simulink model "model"  (R2014a)
(part 4 of 5)

  Ajka___Sümeg_CN_190281225_120000_CN_209328058_120000/RConn2 -- T_209328058__Zalaegerszeg_alállomás/LConn2 -- _CN_312831631_120000_CN_209328058_120000/LConn2
  Ajka___Sümeg_CN_190281225_120000_CN_209328058_120000/RConn3 -- T_209328058__Zalaegerszeg_alállomás/LConn3 -- _CN_312831631_120000_CN_209328058_120000/LConn3 -- bus22/LConn1
  Ajka___Sümeg_CN_190281225_120000_CN_243983151_120000/RConn1 -- T_243983151_120000;11000_Keszthely_alállomás/LConn1 -- Söjtör___Keszthely_CN_243983151_120000_CN_203404634_120000/LConn1 -- Söjtör___Keszthely_CN_243983151_120000_CN_243816689_120000/LConn1 -- Keszthely___Marcali_CN_243983151_120000_CN_311788820_120000/LConn1 -- _CN_243983151_120000_CN_65034002_120000/RConn1 -- _CN_243983151_120000_CN_234435878_120000/LConn1 -- _CN_243983151_120000_CN_170160989_120000/LConn1 -- Keszthely–Hévíz_CN_96705565_120000_CN_243983151_120000/LConn1
  Ajka___Sümeg_CN_190281225_120000_CN_243983151_120000/RConn2 -- T_243983151_120000;11000_Keszthely_alállomás/LConn2 -- Söjtör___Keszthely_CN_243983151_120000_CN_203404634_120000/LConn2 -- Söjtör___Keszthely_CN_243983151_120000_CN_243816689_120000/LConn2 -- Keszthely___Marcali_CN_243983151_120000_CN_311788820_120000/LConn2 -- _CN_243983151_120000_CN_65034002_120000/RConn2 -- _CN_243983151_120000_CN_234435878_120000/LConn2 -- _CN_243983151_120000_CN_170160989_120000/LConn2 -- Keszthely–Hévíz_CN_96705565_120000_CN_243983151_120000/LConn2
  Ajka___Sümeg_CN_190281225_120000_CN_243983151_120000/RConn3 -- T_243983151_120000;11000_Keszthely_alállomás/LConn3 -- Söjtör___Keszthely_CN_243983151_120000_CN_203404634_120000/LConn3 -- Söjtör___Keszthely_CN_243983151_120000_CN_243816689_120000/LConn3 -- bus23/LConn1 -- Keszthely___Marcali_CN_243983151_120000_CN_311788820_120000/LConn3 -- _CN_243983151_120000_CN_65034002_120000/RConn3 -- _CN_243983151_120000_CN_234435878_120000/LConn3 -- _CN_243983151_120000_CN_170160989_120000/LConn3 -- Keszthely–Hévíz_CN_96705565_120000_CN_243983151_120000/LConn3
  T_167473416__/LConn1 -- Ajka___Sümeg_CN_190281225_120000_CN_167473416_120000/RConn1
  T_167473416__/LConn2 -- Ajka___Sümeg_CN_190281225_120000_CN_167473416_120000/RConn2
  Ajka___Sümeg_CN_190281225_120000_CN_167473416_120000/RConn3 -- T_167473416__/LConn3 -- bus24/LConn1
  Ajka___Sümeg_CN_190281225_120000_CN_320532045_120000/RConn1 -- T_320532045__Ajka/LConn1 -- Ajka–Litér_CN_320532045_120000_CN_65034002_120000/RConn1 -- Ikervár___Celldömölk;_Szombathely–Ajka_CN_180089895_120000_CN_320532045_120000/LConn1 -- Pápa–Ajka_CN_320532045_120000_CN_313625037_120000/LConn1
  Ajka___Sümeg_CN_190281225_120000_CN_320532045_120000/RConn2 -- T_320532045__Ajka/LConn2 -- Ajka–Litér_CN_320532045_120000_CN_65034002_120000/RConn2 -- Ikervár___Celldömölk;_Szombathely–Ajka_CN_180089895_120000_CN_320532045_120000/LConn2 -- Pápa–Ajka_CN_320532045_120000_CN_313625037_120000/LConn2
  Ajka___Sümeg_CN_190281225_120000_CN_320532045_120000/RConn3 -- T_320532045__Ajka/LConn3 -- Ajka–Litér_CN_320532045_120000_CN_65034002_120000/RConn3 -- bus25/LConn1 -- Ikervár___Celldömölk;_Szombathely–Ajka_CN_180089895_120000_CN_320532045_120000/LConn3 -- Pápa–Ajka_CN_320532045_120000_CN_313625037_120000/LConn3
  _CN_299594250_120000_CN_299717539_120000/LConn1 -- T_299594250__/LConn1 -- _CN_299594250_120000_CN_301002581_120000/LConn1 -- _CN_299594250_120000_CN_299717558_120000/LConn1
  _CN_299594250_120000_CN_299717539_120000/LConn2 -- T_299594250__/LConn2 -- _CN_299594250_120000_CN_301002581_120000/LConn2 -- _CN_299594250_120000_CN_299717558_120000/LConn2
  _CN_299594250_120000_CN_299717539_120000/LConn3 -- T_299594250__/LConn3 -- _CN_299594250_120000_CN_301002581_120000/LConn3 -- _CN_299594250_120000_CN_299717558_120000/LConn3 -- bus26/LConn1
  _CN_299594250_120000_CN_299717539_120000/RConn1 -- T_299717539__/LConn1 -- _CN_173757619_120000_CN_299717539_120000/LConn1
  _CN_299594250_120000_CN_299717539_120000/RConn2 -- T_299717539__/LConn2 -- _CN_173757619_120000_CN_299717539_120000/LConn2
  _CN_299594250_120000_CN_299717539_120000/RConn3 -- T_299717539__/LConn3 -- _CN_173757619_120000_CN_299717539_120000/LConn3 -- bus27/LConn1
  _CN_299594250_120000_CN_301002581_120000/RConn1 -- T_301002581__/RConn1 -- _CN_104027708_120000_CN_301002581_120000/LConn1 -- Nagybátony_Mátravidéki_Erőmű_CN_173757619_120000_CN_301002581_120000/LConn1 -- L_301002581/LConn1
  _CN_299594250_120000_CN_301002581_120000/RConn2 -- T_301002581__/RConn2 -- _CN_104027708_120000_CN_301002581_120000/LConn2 -- Nagybátony_Mátravidéki_Erőmű_CN_173757619_120000_CN_301002581_120000/LConn2 -- L_301002581/LConn2
  _CN_299594250_120000_CN_301002581_120000/RConn3 -- T_301002581__/RConn3 -- _CN_104027708_120000_CN_301002581_120000/LConn3 -- Nagybátony_Mátravidéki_Erőmű_CN_173757619_120000_CN_301002581_120000/LConn3 -- L_301002581/LConn3 -- bus28/LConn1
  T_299717558__Rétság_alállomás/LConn1 -- _CN_299594250_120000_CN_299717558_120000/RConn1
  T_299717558__Rétság_alállomás/LConn2 -- _CN_299594250_120000_CN_299717558_120000/RConn2
  _CN_299594250_120000_CN_299717558_120000/RConn3 -- T_299717558__Rétság_alállomás/LConn3 -- bus29/LConn1
  Csurgó–Nagyatád_CN_167798796_120000_CN_31538924_120000/LConn1 -- T_167798796__Nagyatád_alállomás/LConn1 -- Csurgó–Nagyatád_CN_167798796_120000_CN_244495956_120000/LConn1 -- Csurgó–Nagyatád_CN_167798796_120000_CN_203404634_120000/LConn1 -- Csurgó–Nagyatád_CN_167798796_120000_CN_121241890_120000/LConn1
  Csurgó–Nagyatád_CN_167798796_120000_CN_31538924_120000/LConn2 -- T_167798796__Nagyatád_alállomás/LConn2 -- Csurgó–Nagyatád_CN_167798796_120000_CN_244495956_120000/LConn2 -- Csurgó–Nagyatád_CN_167798796_120000_CN_203404634_120000/LConn2 -- Csurgó–Nagyatád_CN_167798796_120000_CN_121241890_120000/LConn2
  Csurgó–Nagyatád_CN_167798796_120000_CN_31538924_120000/LConn3 -- T_167798796__Nagyatád_alállomás/LConn3 -- Csurgó–Nagyatád_CN_167798796_120000_CN_244495956_120000/LConn3 -- Csurgó–Nagyatád_CN_167798796_120000_CN_203404634_120000/LConn3 -- bus30/LConn1 -- Csurgó–Nagyatád_CN_167798796_120000_CN_121241890_120000/LConn3
  Csurgó–Nagyatád_CN_167798796_120000_CN_31538924_120000/RConn1 -- T_31538924__Kaposvár_alállomás/LConn1 -- Pécsi_Hőerőmű–(Bonyhád_–_Szekszárd_–_Paks)_Komló_CN_302192173_120000_CN_31538924_120000/LConn1 -- _CN_311788819_120000_CN_31538924_120000/LConn1 -- Kaposvár–Kaposfüred_CN_315669517_120000_CN_31538924_120000/LConn1 -- Kaposvár_–_Sikonda_CN_235409083_120000_CN_31538924_120000/LConn1 -- Kaposvár–Toponár_CN_31538924_120000_CN_113570302_120000/LConn1
  Csurgó–Nagyatád_CN_167798796_120000_CN_31538924_120000/RConn2 -- T_31538924__Kaposvár_alállomás/LConn2 -- Pécsi_Hőerőmű–(Bonyhád_–_Szekszárd_–_Paks)_Komló_CN_302192173_120000_CN_31538924_120000/LConn2 -- _CN_311788819_120000_CN_31538924_120000/LConn2 -- Kaposvár–Kaposfüred_CN_315669517_120000_CN_31538924_120000/LConn2 -- Kaposvár_–_Sikonda_CN_235409083_120000_CN_31538924_120000/LConn2 -- Kaposvár–Toponár_CN_31538924_120000_CN_113570302_120000/LConn2
  Csurgó–Nagyatád_CN_167798796_120000_CN_31538924_120000/RConn3 -- T_31538924__Kaposvár_alállomás/LConn3 -- Pécsi_Hőerőmű–(Bonyhád_–_Szekszárd_–_Paks)_Komló_CN_302192173_120000_CN_31538924_120000/LConn3 -- _CN_311788819_120000_CN_31538924_120000/LConn3 -- Kaposvár–Kaposfüred_CN_315669517_120000_CN_31538924_120000/LConn3 -- Kaposvár_–_Sikonda_CN_235409083_120000_CN_31538924_120000/LConn3 -- Kaposvár–Toponár_CN_31538924_120000_CN_113570302_120000/LConn3 -- bus31/LConn1
  Csurgó–Nagyatád_CN_167798796_120000_CN_121241890_120000/RConn1 -- T_121241890__Szigetvár_120_kV_alállomás/LConn1 -- Kővágószőlős–Szigetvár_CN_121241890_120000_CN_313889220_120000/LConn1 -- Barcs___Szigetvár_120_Kv_s_távvezeték_CN_121241890_120000_CN_121135019_120000/LConn1
  Csurgó–Nagyatád_CN_167798796_120000_CN_121241890_120000/RConn2 -- T_121241890__Szigetvár_120_kV_alállomás/LConn2 -- Kővágószőlős–Szigetvár_CN_121241890_120000_CN_313889220_120000/LConn2 -- Barcs___Szigetvár_120_Kv_s_távvezeték_CN_121241890_120000_CN_121135019_120000/LConn2
  Csurgó–Nagyatád_CN_167798796_120000_CN_121241890_120000/RConn3 -- T_121241890__Szigetvár_120_kV_alállomás/LConn3 -- Kővágószőlős–Szigetvár_CN_121241890_120000_CN_313889220_120000/LConn3 -- bus32/LConn1 -- Barcs___Szigetvár_120_Kv_s_távvezeték_CN_121241890_120000_CN_121135019_120000/LConn3
  T_244495956__Csurgó_alállomás/LConn1 -- Csurgó–Nagyatád_CN_167798796_120000_CN_244495956_120000/RConn1
  T_244495956__Csurgó_alállomás/LConn2 -- Csurgó–Nagyatád_CN_167798796_120000_CN_244495956_120000/RConn2
  Csurgó–Nagyatád_CN_167798796_120000_CN_244495956_120000/RConn3 -- T_244495956__Csurgó_alállomás/LConn3 -- bus33/LConn1
  Csurgó–Nagyatád_CN_167798796_120000_CN_203404634_120000/RConn1 -- T_203404634_120000;20000;10000_Nagykanizsa_alállomás/LConn1 -- Söjtör___Keszthely_CN_243983151_120000_CN_203404634_120000/RConn1 -- Kanizsavár___Nagykanizsa_CN_203404634_120000_CN_243726196_120000/LConn1
  Csurgó–Nagyatád_CN_167798796_120000_CN_203404634_120000/RConn2 -- T_203404634_120000;20000;10000_Nagykanizsa_alállomás/LConn2 -- Söjtör___Keszthely_CN_243983151_120000_CN_203404634_120000/RConn2 -- Kanizsavár___Nagykanizsa_CN_203404634_120000_CN_243726196_120000/LConn2
  Csurgó–Nagyatád_CN_167798796_120000_CN_203404634_120000/RConn3 -- T_203404634_120000;20000;10000_Nagykanizsa_alállomás/LConn3 -- Söjtör___Keszthely_CN_243983151_120000_CN_203404634_120000/RConn3 -- Kanizsavár___Nagykanizsa_CN_203404634_120000_CN_243726196_120000/LConn3 -- bus34/LConn1
  _CN_254851597_120000_CN_254847446_120000/LConn1 -- T_254851597__Bicske_alállomás/LConn1 -- _CN_254851597_120000_CN_254910050_120000/RConn1
  _CN_254851597_120000_CN_254847446_120000/LConn2 -- T_254851597__Bicske_alállomás/LConn2 -- _CN_254851597_120000_CN_254910050_120000/RConn2
  _CN_254851597_120000_CN_254847446_120000/LConn3 -- T_254851597__Bicske_alállomás/LConn3 -- _CN_254851597_120000_CN_254910050_120000/RConn3 -- bus35/LConn1
  _CN_254851597_120000_CN_254847446_120000/RConn1 -- T_254847446__Bicske_dél_alállomás/RConn1 -- _CN_153098964_120000_CN_254847446_120000/LConn1 -- L_254847446/LConn1
  _CN_254851597_120000_CN_254847446_120000/RConn2 -- T_254847446__Bicske_dél_alállomás/RConn2 -- _CN_153098964_120000_CN_254847446_120000/LConn2 -- L_254847446/LConn2
  _CN_254851597_120000_CN_254847446_120000/RConn3 -- T_254847446__Bicske_dél_alállomás/RConn3 -- _CN_153098964_120000_CN_254847446_120000/LConn3 -- L_254847446/LConn3 -- bus36/LConn1
  T_350686736__Győr_Dunapart_alállomás/LConn1 -- _CN_350686736_120000_CN_350230665_120000/LConn1
  T_350686736__Győr_Dunapart_alállomás/LConn2 -- _CN_350686736_120000_CN_350230665_120000/LConn2
  _CN_350686736_120000_CN_350230665_120000/LConn3 -- T_350686736__Győr_Dunapart_alállomás/LConn3 -- bus37/LConn1
  _CN_350686736_120000_CN_350230665_120000/RConn1 -- T_350230665__Győr_ÉDÁSZ_alállomás/LConn1 -- _CN_124244078_120000_CN_350230665_120000/LConn1 -- _CN_267155016_120000_CN_350230665_120000/LConn1
  _CN_350686736_120000_CN_350230665_120000/RConn2 -- T_350230665__Győr_ÉDÁSZ_alállomás/LConn2 -- _CN_124244078_120000_CN_350230665_120000/LConn2 -- _CN_267155016_120000_CN_350230665_120000/LConn2
  _CN_350686736_120000_CN_350230665_120000/RConn3 -- T_350230665__Győr_ÉDÁSZ_alállomás/LConn3 -- _CN_124244078_120000_CN_350230665_120000/LConn3 -- bus38/LConn1 -- _CN_267155016_120000_CN_350230665_120000/LConn3
  T_288399377__Szeged_Cserepes_sori_alállomás/LConn1 -- _CN_288399377_120000_CN_111678830_120000/LConn1
  T_288399377__Szeged_Cserepes_sori_alállomás/LConn2 -- _CN_288399377_120000_CN_111678830_120000/LConn2
  _CN_288399377_120000_CN_111678830_120000/LConn3 -- T_288399377__Szeged_Cserepes_sori_alállomás/LConn3 -- bus39/LConn1
  _CN_288399377_120000_CN_111678830_120000/RConn1 -- T_111678830__Szeged_alállomás/RConn1 -- Szeged___Sándorfalva_CN_100962927_120000_CN_111678830_120000/LConn1 -- L_111678830/LConn1
  _CN_288399377_120000_CN_111678830_120000/RConn2 -- T_111678830__Szeged_alállomás/RConn2 -- Szeged___Sándorfalva_CN_100962927_120000_CN_111678830_120000/LConn2 -- L_111678830/LConn2
  _CN_288399377_120000_CN_111678830_120000/RConn3 -- T_111678830__Szeged_alállomás/RConn3 -- Szeged___Sándorfalva_CN_100962927_120000_CN_111678830_120000/LConn3 -- L_111678830/LConn3 -- bus40/LConn1
  T_296680978__/LConn1 -- _CN_296680978_120000_CN_119367515_120000/LConn1
  T_296680978__/LConn2 -- _CN_296680978_120000_CN_119367515_120000/LConn2
  _CN_296680978_120000_CN_119367515_120000/LConn3 -- T_296680978__/LConn3 -- bus41/LConn1
  T_119367515__/LConn1 -- _CN_296680978_120000_CN_119367515_120000/RConn1
  T_119367515__/LConn2 -- _CN_296680978_120000_CN_119367515_120000/RConn2
  _CN_296680978_120000_CN_119367515_120000/RConn3 -- T_119367515__/LConn3 -- bus42/LConn1
  T_251991299_220000;120000_Detk_220_120_kV_os_alállomás/LConn1 -- Nagybátony___Detk_CN_251991299_120000_CN_173757619_120000/LConn1
  T_251991299_220000;120000_Detk_220_120_kV_os_alállomás/LConn2 -- Nagybátony___Detk_CN_251991299_120000_CN_173757619_120000/LConn2
  Nagybátony___Detk_CN_251991299_120000_CN_173757619_120000/LConn3 -- T_251991299_220000;120000_Detk_220_120_kV_os_alállomás/LConn3 -- bus43/LConn1
  Nagybátony___Detk_CN_251991299_120000_CN_173757619_120000/RConn1 -- T_173757619__Nagybátony_alállomás/LConn1 -- _CN_173757619_120000_CN_299717539_120000/RConn1 -- Salgótarján_Öntöde_–_Nagybátony_CN_173757619_120000_CN_355349327_120000/LConn1 -- Nagybátony_Mátravidéki_Erőmű_CN_173757619_120000_CN_301002581_120000/RConn1 -- Nagybátony___Borsodnádasd_CN_173757619_120000_CN_302147975_120000/LConn1
  Nagybátony___Detk_CN_251991299_120000_CN_173757619_120000/RConn2 -- T_173757619__Nagybátony_alállomás/LConn2 -- _CN_173757619_120000_CN_299717539_120000/RConn2 -- Salgótarján_Öntöde_–_Nagybátony_CN_173757619_120000_CN_355349327_120000/LConn2 -- Nagybátony_Mátravidéki_Erőmű_CN_173757619_120000_CN_301002581_120000/RConn2 -- Nagybátony___Borsodnádasd_CN_173757619_120000_CN_302147975_120000/LConn2
  Nagybátony___Detk_CN_251991299_120000_CN_173757619_120000/RConn3 -- T_173757619__Nagybátony_alállomás/LConn3 -- _CN_173757619_120000_CN_299717539_120000/RConn3 -- Salgótarján_Öntöde_–_Nagybátony_CN_173757619_120000_CN_355349327_120000/LConn3 -- Nagybátony_Mátravidéki_Erőmű_CN_173757619_120000_CN_301002581_120000/RConn3 -- bus44/LConn1 -- Nagybátony___Borsodnádasd_CN_173757619_120000_CN_302147975_120000/LConn3
  T_299574805__/LConn1 -- _CN_299574805_120000_CN_252028146_120000/LConn1
  T_299574805__/LConn2 -- _CN_299574805_120000_CN_252028146_120000/LConn2
  _CN_299574805_120000_CN_252028146_120000/LConn3 -- T_299574805__/LConn3 -- bus45/LConn1
  _CN_299574805_120000_CN_252028146_120000/RConn1 -- T_252028146_220000;120000;12000_Szolnok_220_120_20_kV_os_Alállomás/RConn4 -- _CN_252028146_120000_CN_289011848_120000/LConn1 -- _CN_252028146_120000_CN_288863210_120000/LConn1 -- L_252028146/LConn1 -- Tiszakécske–Városföld_CN_281553159_120000_CN_252028146_120000/LConn1 -- _CN_321513575_120000_CN_252028146_120000/LConn1 -- Szolnok–Cegléd_CN_223956685_120000_CN_252028146_120000/LConn1
  _CN_299574805_120000_CN_252028146_120000/RConn2 -- T_252028146_220000;120000;12000_Szolnok_220_120_20_kV_os_Alállomás/RConn5 -- _CN_252028146_120000_CN_289011848_120000/LConn2 -- _CN_252028146_120000_CN_288863210_120000/LConn2 -- L_252028146/LConn2 -- Tiszakécske–Városföld_CN_281553159_120000_CN_252028146_120000/LConn2 -- _CN_321513575_120000_CN_252028146_120000/LConn2 -- Szolnok–Cegléd_CN_223956685_120000_CN_252028146_120000/LConn2
  _CN_299574805_120000_CN_252028146_120000/RConn3 -- T_252028146_220000;120000;12000_Szolnok_220_120_20_kV_os_Alállomás/RConn6 -- _CN_252028146_120000_CN_289011848_120000/LConn3 -- _CN_252028146_120000_CN_288863210_120000/LConn3 -- L_252028146/LConn3 -- bus46/LConn1 -- Tiszakécske–Városföld_CN_281553159_120000_CN_252028146_120000/LConn3 -- _CN_321513575_120000_CN_252028146_120000/LConn3 -- Szolnok–Cegléd_CN_223956685_120000_CN_252028146_120000/LConn3
  Keszthely–Hévíz_CN_96705565_120000_CN_243983151_120000/RConn1 -- T_96705565_400000;120000_Hévíz_400_120_kV_alállomás/RConn1 -- L_96705565/LConn1
  Keszthely–Hévíz_CN_96705565_120000_CN_243983151_120000/RConn2 -- T_96705565_400000;120000_Hévíz_400_120_kV_alállomás/RConn2 -- L_96705565/LConn2
  Keszthely–Hévíz_CN_96705565_120000_CN_243983151_120000/RConn3 -- T_96705565_400000;120000_Hévíz_400_120_kV_alállomás/RConn3 -- L_96705565/LConn3 -- bus47/LConn1
  T_351673886__/LConn1 -- _CN_351673886_120000_CN_313889220_120000/LConn1
  T_351673886__/LConn2 -- _CN_351673886_120000_CN_313889220_120000/LConn2
  _CN_351673886_120000_CN_313889220_120000/LConn3 -- T_351673886__/LConn3 -- bus48/LConn1
  _CN_351673886_120000_CN_313889220_120000/RConn1 -- T_313889220__Kővágószőlős_alállomás/LConn1 -- Kővágószőlős–Szigetvár_CN_121241890_120000_CN_313889220_120000/RConn1 -- Kővágószőlős–Pécs_Újmecsekalja_CN_293373698_120000_CN_313889220_120000/LConn1
  _CN_351673886_120000_CN_313889220_120000/RConn2 -- T_313889220__Kővágószőlős_alállomás/LConn2 -- Kővágószőlős–Szigetvár_CN_121241890_120000_CN_313889220_120000/RConn2 -- Kővágószőlős–Pécs_Újmecsekalja_CN_293373698_120000_CN_313889220_120000/LConn2
  _CN_351673886_120000_CN_313889220_120000/RConn3 -- T_313889220__Kővágószőlős_alállomás/LConn3 -- Kővágószőlős–Szigetvár_CN_121241890_120000_CN_313889220_120000/RConn3 -- bus49/LConn1 -- Kővágószőlős–Pécs_Újmecsekalja_CN_293373698_120000_CN_313889220_120000/LConn3
  _CN_285319199_120000_CN_285317363_120000/LConn1 -- T_285319199__/RConn1 -- L_285319199/LConn1
  _CN_285319199_120000_CN_285317363_120000/LConn2 -- T_285319199__/RConn2 -- L_285319199/LConn2
  _CN_285319199_120000_CN_285317363_120000/LConn3 -- T_285319199__/RConn3 -- L_285319199/LConn3 -- bus50/LConn1
  _CN_285319199_120000_CN_285317363_120000/RConn1 -- T_285317363__/LConn1 -- Sándorfalva___Kiskunfélegyháza_CN_100962927_120000_CN_285317363_120000/LConn1
  _CN_285319199_120000_CN_285317363_120000/RConn2 -- T_285317363__/LConn2 -- Sándorfalva___Kiskunfélegyháza_CN_100962927_120000_CN_285317363_120000/LConn2
  _CN_285319199_120000_CN_285317363_120000/RConn3 -- T_285317363__/LConn3 -- Sándorfalva___Kiskunfélegyháza_CN_100962927_120000_CN_285317363_120000/LConn3 -- bus51/LConn1
  Tiszakécske–Városföld_CN_281553159_120000_CN_153827138_120000/LConn1 -- T_281553159__Tiszakécske/LConn1 -- Tiszakécske–Városföld_CN_281553159_120000_CN_252028146_120000/RConn1
  Tiszakécske–Városföld_CN_281553159_120000_CN_153827138_120000/LConn2 -- T_281553159__Tiszakécske/LConn2 -- Tiszakécske–Városföld_CN_281553159_120000_CN_252028146_120000/RConn2
  Tiszakécske–Városföld_CN_281553159_120000_CN_153827138_120000/LConn3 -- T_281553159__Tiszakécske/LConn3 -- Tiszakécske–Városföld_CN_281553159_120000_CN_252028146_120000/RConn3 -- bus52/LConn1
  Tiszakécske–Városföld_CN_281553159_120000_CN_153827138_120000/RConn1 -- T_153827138__Városföld_alállomás/LConn1 -- _CN_153827138_120000_CN_283021123_120000/LConn1 -- _CN_153827138_120000_CN_280595113_120000/LConn1 -- Cegléd–Nagykőrös_CN_223956685_120000_CN_153827138_120000/LConn1
  Tiszakécske–Városföld_CN_281553159_120000_CN_153827138_120000/RConn2 -- T_153827138__Városföld_alállomás/LConn2 -- _CN_153827138_120000_CN_283021123_120000/LConn2 -- _CN_153827138_120000_CN_280595113_120000/LConn2 -- Cegléd–Nagykőrös_CN_223956685_120000_CN_153827138_120000/LConn2
  Tiszakécske–Városföld_CN_281553159_120000_CN_153827138_120000/RConn3 -- T_153827138__Városföld_alállomás/LConn3 -- _CN_153827138_120000_CN_283021123_120000/LConn3 -- _CN_153827138_120000_CN_280595113_120000/LConn3 -- bus53/LConn1 -- Cegléd–Nagykőrös_CN_223956685_120000_CN_153827138_120000/LConn3
  _CN_289183579_120000_CN_289183615_120000/LConn1 -- T_289183579__/LConn1 -- _CN_289183579_120000_CN_288863087_120000/LConn1
  _CN_289183579_120000_CN_289183615_120000/LConn2 -- T_289183579__/LConn2 -- _CN_289183579_120000_CN_288863087_120000/LConn2
  _CN_289183579_120000_CN_289183615_120000/LConn3 -- T_289183579__/LConn3 -- _CN_289183579_120000_CN_288863087_120000/LConn3 -- bus54/LConn1
  _CN_289183579_120000_CN_289183615_120000/RConn1 -- T_289183615__/LConn1 -- _CN_251018027_120000_CN_289183615_120000/LConn1
  _CN_289183579_120000_CN_289183615_120000/RConn2 -- T_289183615__/LConn2 -- _CN_251018027_120000_CN_289183615_120000/LConn2
  _CN_289183579_120000_CN_289183615_120000/RConn3 -- T_289183615__/LConn3 -- _CN_251018027_120000_CN_289183615_120000/LConn3 -- bus55/LConn1
  _CN_289183579_120000_CN_288863087_120000/RConn1 -- T_288863087__Mezőtúr_120_kV_alállomás/LConn1 -- _CN_288864314_120000_CN_288863087_120000/LConn1 -- Mezőtúr___Békéscsaba_CN_288863087_120000_CN_287201135_120000/LConn1
  _CN_289183579_120000_CN_288863087_120000/RConn2 -- T_288863087__Mezőtúr_120_kV_alállomás/LConn2 -- _CN_288864314_120000_CN_288863087_120000/LConn2 -- Mezőtúr___Békéscsaba_CN_288863087_120000_CN_287201135_120000/LConn2
  _CN_289183579_120000_CN_288863087_120000/RConn3 -- T_288863087__Mezőtúr_120_kV_alállomás/LConn3 -- _CN_288864314_120000_CN_288863087_120000/LConn3 -- Mezőtúr___Békéscsaba_CN_288863087_120000_CN_287201135_120000/LConn3 -- bus56/LConn1
  T_121661769_120000_/LConn1 -- _CN_103952390_120000_CN_121661769_120000/RConn1
  T_121661769_120000_/LConn2 -- _CN_103952390_120000_CN_121661769_120000/RConn2
  _CN_103952390_120000_CN_121661769_120000/RConn3 -- T_121661769_120000_/LConn3 -- bus57/LConn1
  _CN_103952390_120000_CN_136396751_120000/RConn1 -- T_136396751__Hüvösvölgy_alállomás/LConn1 -- _CN_153098964_120000_CN_136396751_120000/LConn1
  _CN_103952390_120000_CN_136396751_120000/RConn2 -- T_136396751__Hüvösvölgy_alállomás/LConn2 -- _CN_153098964_120000_CN_136396751_120000/LConn2
  _CN_103952390_120000_CN_136396751_120000/RConn3 -- T_136396751__Hüvösvölgy_alállomás/LConn3 -- _CN_153098964_120000_CN_136396751_120000/LConn3 -- bus58/LConn1
  Kaszásdűlő___Pomáz_CN_103952390_120000_CN_252727452_120000/RConn1 -- T_252727452_120000_Pomáz/LConn1 -- _CN_209157413_120000_CN_252727452_120000/LConn1
  Kaszásdűlő___Pomáz_CN_103952390_120000_CN_252727452_120000/RConn2 -- T_252727452_120000_Pomáz/LConn2 -- _CN_209157413_120000_CN_252727452_120000/LConn2
  Kaszásdűlő___Pomáz_CN_103952390_120000_CN_252727452_120000/RConn3 -- T_252727452_120000_Pomáz/LConn3 -- _CN_209157413_120000_CN_252727452_120000/LConn3 -- bus59/LConn1
  Kaszásdűlő___Pomáz_CN_103952390_120000_CN_100872886_120000/RConn1 -- T_100872886__Göd_alállomás/RConn4 -- _CN_253313109_120000_CN_100872886_120000/LConn1 -- _CN_252610696_120000_CN_100872886_120000/RConn1 -- _CN_100872886_120000_CN_103950678_120000/LConn1 -- _CN_100872886_120000_CN_103950687_120000/LConn1 -- L_100872886/LConn1
  Kaszásdűlő___Pomáz_CN_103952390_120000_CN_100872886_120000/RConn2 -- T_100872886__Göd_alállomás/RConn5 -- _CN_253313109_120000_CN_100872886_120000/LConn2 -- _CN_252610696_120000_CN_100872886_120000/RConn2 -- _CN_100872886_120000_CN_103950678_120000/LConn2 -- _CN_100872886_120000_CN_103950687_120000/LConn2 -- L_100872886/LConn2
  Kaszásdűlő___Pomáz_CN_103952390_120000_CN_100872886_120000/RConn3 -- T_100872886__Göd_alállomás/RConn6 -- _CN_253313109_120000_CN_100872886_120000/LConn3 -- _CN_252610696_120000_CN_100872886_120000/RConn3 -- _CN_100872886_120000_CN_103950678_120000/LConn3 -- _CN_100872886_120000_CN_103950687_120000/LConn3 -- L_100872886/LConn3 -- bus60/LConn1
  T_116801424_120000_Békásmegyer/LConn1 -- Kaszásdűlő___Pomáz_CN_103952390_120000_CN_116801424_120000/RConn1
  T_116801424_120000_Békásmegyer/LConn2 -- Kaszásdűlő___Pomáz_CN_103952390_120000_CN_116801424_120000/RConn2
  Kaszásdűlő___Pomáz_CN_103952390_120000_CN_116801424_120000/RConn3 -- T_116801424_120000_Békásmegyer/LConn3 -- bus61/LConn1
  Ikervár___Celldömölk;_Szombathely–Ajka_CN_180089895_120000_CN_302056631_120000/LConn1 -- T_180089895__Celldömölk/LConn1 -- Ikervár___Celldömölk;_Szombathely–Ajka_CN_180089895_120000_CN_320532045_120000/RConn1 -- Ikervár___Celldömölk;_Szombathely–Ajka_CN_180089895_120000_CN_245836377_120000/LConn1
  Ikervár___Celldömölk;_Szombathely–Ajka_CN_180089895_120000_CN_302056631_120000/LConn2 -- T_180089895__Celldömölk/LConn2 -- Ikervár___Celldömölk;_Szombathely–Ajka_CN_180089895_120000_CN_320532045_120000/RConn2 -- Ikervár___Celldömölk;_Szombathely–Ajka_CN_180089895_120000_CN_245836377_120000/LConn2
  Ikervár___Celldömölk;_Szombathely–Ajka_CN_180089895_120000_CN_302056631_120000/LConn3 -- T_180089895__Celldömölk/LConn3 -- Ikervár___Celldömölk;_Szombathely–Ajka_CN_180089895_120000_CN_320532045_120000/RConn3 -- bus62/LConn1 -- Ikervár___Celldömölk;_Szombathely–Ajka_CN_180089895_120000_CN_245836377_120000/LConn3
  T_302056631__Ikervár_alállomás/LConn1 -- Ikervár___Celldömölk;_Szombathely–Ajka_CN_180089895_120000_CN_302056631_120000/RConn1
  T_302056631__Ikervár_alállomás/LConn2 -- Ikervár___Celldömölk;_Szombathely–Ajka_CN_180089895_120000_CN_302056631_120000/RConn2
  Ikervár___Celldömölk;_Szombathely–Ajka_CN_180089895_120000_CN_302056631_120000/RConn3 -- T_302056631__Ikervár_alállomás/LConn3 -- bus63/LConn1
  Ikervár___Celldömölk;_Szombathely–Ajka_CN_180089895_120000_CN_245836377_120000/RConn1 -- T_245836377_120000_Szombathely_120_kV_alállomás/LConn1 -- _CN_245836377_120000_CN_166155511_120000/LConn1 -- _CN_245836377_120000_CN_178641777_120000/LConn1 -- _CN_245836377_120000_CN_312831631_120000/LConn1 -- _CN_245836377_120000_CN_204596172_120000/LConn1
  Ikervár___Celldömölk;_Szombathely–Ajka_CN_180089895_120000_CN_245836377_120000/RConn2 -- T_245836377_120000_Szombathely_120_kV_alállomás/LConn2 -- _CN_245836377_120000_CN_166155511_120000/LConn2 -- _CN_245836377_120000_CN_178641777_120000/LConn2 -- _CN_245836377_120000_CN_312831631_120000/LConn2 -- _CN_245836377_120000_CN_204596172_120000/LConn2
  Ikervár___Celldömölk;_Szombathely–Ajka_CN_180089895_120000_CN_245836377_120000/RConn3 -- T_245836377_120000_Szombathely_120_kV_alállomás/LConn3 -- _CN_245836377_120000_CN_166155511_120000/LConn3 -- _CN_245836377_120000_CN_178641777_120000/LConn3 -- _CN_245836377_120000_CN_312831631_120000/LConn3 -- bus64/LConn1 -- _CN_245836377_120000_CN_204596172_120000/LConn3
  Nyíregyháza_MÁV_II_CN_292353065_120000_CN_292353077_120000/LConn1 -- T_292353065__MÁV_120_25kV/LConn1 -- Nyíregyháza_MÁV_II_CN_292353065_120000_CN_229990586_120000/LConn1
  Nyíregyháza_MÁV_II_CN_292353065_120000_CN_292353077_120000/LConn2 -- T_292353065__MÁV_120_25kV/LConn2 -- Nyíregyháza_MÁV_II_CN_292353065_120000_CN_229990586_120000/LConn2
  Nyíregyháza_MÁV_II_CN_292353065_120000_CN_292353077_120000/LConn3 -- T_292353065__MÁV_120_25kV/LConn3 -- Nyíregyháza_MÁV_II_CN_292353065_120000_CN_229990586_120000/LConn3 -- bus65/LConn1
  Nyíregyháza_MÁV_II_CN_292353065_120000_CN_292353077_120000/RConn1 -- T_292353077__Simai_úti_120_20kV/LConn1 -- Tiszalök_Nyíregyháza_CN_292353077_120000_CN_251018027_120000/LConn1 -- _CN_250030343_120000_CN_292353077_120000/LConn1 -- Kisvárda_–_Nyíregyháza_CN_292353077_120000_CN_289912792_120000/LConn1
  Nyíregyháza_MÁV_II_CN_292353065_120000_CN_292353077_120000/RConn2 -- T_292353077__Simai_úti_120_20kV/LConn2 -- Tiszalök_Nyíregyháza_CN_292353077_120000_CN_251018027_120000/LConn2 -- _CN_250030343_120000_CN_292353077_120000/LConn2 -- Kisvárda_–_Nyíregyháza_CN_292353077_120000_CN_289912792_120000/LConn2
  Nyíregyháza_MÁV_II_CN_292353065_120000_CN_292353077_120000/RConn3 -- T_292353077__Simai_úti_120_20kV/LConn3 -- Tiszalök_Nyíregyháza_CN_292353077_120000_CN_251018027_120000/LConn3 -- bus66/LConn1 -- _CN_250030343_120000_CN_292353077_120000/LConn3 -- Kisvárda_–_Nyíregyháza_CN_292353077_120000_CN_289912792_120000/LConn3
  T_229990586_120000;10000_Nyíregyháza_Dél/LConn1 -- Nyíregyháza_MÁV_II_CN_292353065_120000_CN_229990586_120000/RConn1
  T_229990586_120000;10000_Nyíregyháza_Dél/LConn2 -- Nyíregyháza_MÁV_II_CN_292353065_120000_CN_229990586_120000/RConn2
  Nyíregyháza_MÁV_II_CN_292353065_120000_CN_229990586_120000/RConn3 -- T_229990586_120000;10000_Nyíregyháza_Dél/LConn3 -- bus67/LConn1
  T_250030343__Ibrány/LConn1 -- _CN_250030343_120000_CN_292353077_120000/RConn1
  T_250030343__Ibrány/LConn2 -- _CN_250030343_120000_CN_292353077_120000/RConn2
  _CN_250030343_120000_CN_292353077_120000/RConn3 -- T_250030343__Ibrány/LConn3 -- bus68/LConn1
  Pécs_Újmecsekalja–Pécsi_Hőerőmű_CN_302192173_120000_CN_293373698_120000/LConn1 -- T_302192173__/LConn1 -- Pécs_Kelet–Pécsi_Hőerőmű_CN_302192173_120000_CN_33846555_120000/LConn1 -- Pécsi_Hőerőmű–(Bonyhád_–_Szekszárd_–_Paks)_Komló_CN_302192173_120000_CN_121501391_120000/LConn1 -- Pécsi_Hőerőmű–(Bonyhád_–_Szekszárd_–_Paks)_Komló_CN_302192173_120000_CN_336632820_120000/LConn1 -- Pécsi_Hőerőmű–(Bonyhád_–_Szekszárd_–_Paks)_Komló_CN_302192173_120000_CN_100788162_120000/LConn1 -- Pécsi_Hőerőmű–(Bonyhád_–_Szekszárd_–_Paks)_Komló_CN_302192173_120000_CN_31538924_120000/RConn1 -- Pécsi_Hőerőmű_–_Komló_CN_302192173_120000_CN_331140850_120000/LConn1 -- Pécsi_Hőerőmű–Mohács_CN_302192173_120000_CN_156193065_120000/LConn1 -- Pécs_Újmecsekalja–Pécsi_Hőerőmű_CN_302192173_120000_CN_254787562_120000/LConn1 -- Pécsi_Hőerőmű–Siklós_CN_302192173_120000_CN_315839275_120000/LConn1 -- Pécsi_Hőerőmű–Siklós_CN_302192173_120000_CN_315953570_120000/LConn1
  Pécs_Újmecsekalja–Pécsi_Hőerőmű_CN_302192173_120000_CN_293373698_120000/LConn2 -- T_302192173__/LConn2 -- Pécs_Kelet–Pécsi_Hőerőmű_CN_302192173_120000_CN_33846555_120000/LConn2 -- Pécsi_Hőerőmű–(Bonyhád_–_Szekszárd_–_Paks)_Komló_CN_302192173_120000_CN_121501391_120000/LConn2 -- Pécsi_Hőerőmű–(Bonyhád_–_Szekszárd_–_Paks)_Komló_CN_302192173_120000_CN_336632820_120000/LConn2 -- Pécsi_Hőerőmű–(Bonyhád_–_Szekszárd_–_Paks)_Komló_CN_302192173_120000_CN_100788162_120000/LConn2 -- Pécsi_Hőerőmű–(Bonyhád_–_Szekszárd_–_Paks)_Komló_CN_302192173_120000_CN_31538924_120000/RConn2 -- Pécsi_Hőerőmű_–_Komló_CN_302192173_120000_CN_331140850_120000/LConn2 -- Pécsi_Hőerőmű–Mohács_CN_302192173_120000_CN_156193065_120000/LConn2 -- Pécs_Újmecsekalja–Pécsi_Hőerőmű_CN_302192173_120000_CN_254787562_120000/LConn2 -- Pécsi_Hőerőmű–Siklós_CN_302192173_120000_CN_315839275_120000/LConn2 -- Pécsi_Hőerőmű–Siklós_CN_302192173_120000_CN_315953570_120000/LConn2
  Pécs_Újmecsekalja–Pécsi_Hőerőmű_CN_302192173_120000_CN_293373698_120000/LConn3 -- T_302192173__/LConn3 -- Pécs_Kelet–Pécsi_Hőerőmű_CN_302192173_120000_CN_33846555_120000/LConn3 -- Pécsi_Hőerőmű–(Bonyhád_–_Szekszárd_–_Paks)_Komló_CN_302192173_120000_CN_121501391_120000/LConn3 -- Pécsi_Hőerőmű–(Bonyhád_–_Szekszárd_–_Paks)_Komló_CN_302192173_120000_CN_336632820_120000/LConn3 -- Pécsi_Hőerőmű–(Bonyhád_–_Szekszárd_–_Paks)_Komló_CN_302192173_120000_CN_100788162_120000/LConn3 -- Pécsi_Hőerőmű–(Bonyhád_–_Szekszárd_–_Paks)_Komló_CN_302192173_120000_CN_31538924_120000/RConn3 -- Pécsi_Hőerőmű_–_Komló_CN_302192173_120000_CN_331140850_120000/LConn3 -- Pécsi_Hőerőmű–Mohács_CN_302192173_120000_CN_156193065_120000/LConn3 -- bus69/LConn1 -- Pécs_Újmecsekalja–Pécsi_Hőerőmű_CN_302192173_120000_CN_254787562_120000/LConn3 -- Pécsi_Hőerőmű–Siklós_CN_302192173_120000_CN_315839275_120000/LConn3 -- Pécsi_Hőerőmű–Siklós_CN_302192173_120000_CN_315953570_120000/LConn3
  Pécs_Újmecsekalja–Pécsi_Hőerőmű_CN_302192173_120000_CN_293373698_120000/RConn1 -- T_293373698__Pécs_Újmecsekalja_alállomás/LConn1 -- Kővágószőlős–Pécs_Újmecsekalja_CN_293373698_120000_CN_313889220_120000/RConn1
  Pécs_Újmecsekalja–Pécsi_Hőerőmű_CN_302192173_120000_CN_293373698_120000/RConn2 -- T_293373698__Pécs_Újmecsekalja_alállomás/LConn2 -- Kővágószőlős–Pécs_Újmecsekalja_CN_293373698_120000_CN_313889220_120000/RConn2
  Pécs_Újmecsekalja–Pécsi_Hőerőmű_CN_302192173_120000_CN_293373698_120000/RConn3 -- T_293373698__Pécs_Újmecsekalja_alállomás/LConn3 -- Kővágószőlős–Pécs_Újmecsekalja_CN_293373698_120000_CN_313889220_120000/RConn3 -- bus70/LConn1
  T_254787562__Pécs_Kertváros_alállomás/LConn1 -- Pécs_Újmecsekalja–Pécsi_Hőerőmű_CN_302192173_120000_CN_254787562_120000/RConn1
  T_254787562__Pécs_Kertváros_alállomás/LConn2 -- Pécs_Újmecsekalja–Pécsi_Hőerőmű_CN_302192173_120000_CN_254787562_120000/RConn2
  Pécs_Újmecsekalja–Pécsi_Hőerőmű_CN_302192173_120000_CN_254787562_120000/RConn3 -- T_254787562__Pécs_Kertváros_alállomás/LConn3 -- bus71/LConn1
  T_315839275__Siklós_alállomás/LConn1 -- Pécsi_Hőerőmű–Siklós_CN_302192173_120000_CN_315839275_120000/RConn1
  T_315839275__Siklós_alállomás/LConn2 -- Pécsi_Hőerőmű–Siklós_CN_302192173_120000_CN_315839275_120000/RConn2
  Pécsi_Hőerőmű–Siklós_CN_302192173_120000_CN_315839275_120000/RConn3 -- T_315839275__Siklós_alállomás/LConn3 -- bus72/LConn1
  T_315953570__/LConn1 -- Pécsi_Hőerőmű–Siklós_CN_302192173_120000_CN_315953570_120000/RConn1
  T_315953570__/LConn2 -- Pécsi_Hőerőmű–Siklós_CN_302192173_120000_CN_315953570_120000/RConn2
  Pécsi_Hőerőmű–Siklós_CN_302192173_120000_CN_315953570_120000/RConn3 -- T_315953570__/LConn3 -- bus73/LConn1
  Pécs_Kelet–Pécsi_Hőerőmű_CN_302192173_120000_CN_33846555_120000/RConn1 -- T_33846555_400000;120000_Pécs_Kelet_alállomás/RConn1 -- L_33846555/LConn1
  Pécs_Kelet–Pécsi_Hőerőmű_CN_302192173_120000_CN_33846555_120000/RConn2 -- T_33846555_400000;120000_Pécs_Kelet_alállomás/RConn2 -- L_33846555/LConn2
  Pécs_Kelet–Pécsi_Hőerőmű_CN_302192173_120000_CN_33846555_120000/RConn3 -- T_33846555_400000;120000_Pécs_Kelet_alállomás/RConn3 -- L_33846555/LConn3 -- bus74/LConn1
  Pécsi_Hőerőmű–(Bonyhád_–_Szekszárd_–_Paks)_Komló_CN_302192173_120000_CN_121501391_120000/RConn1 -- T_121501391__Komló_alállomás/LConn1 -- Komló_–_Sikonda_CN_235409083_120000_CN_121501391_120000/LConn1
  Pécsi_Hőerőmű–(Bonyhád_–_Szekszárd_–_Paks)_Komló_CN_302192173_120000_CN_121501391_120000/RConn2 -- T_121501391__Komló_alállomás/LConn2 -- Komló_–_Sikonda_CN_235409083_120000_CN_121501391_120000/LConn2
  Pécsi_Hőerőmű–(Bonyhád_–_Szekszárd_–_Paks)_Komló_CN_302192173_120000_CN_121501391_120000/RConn3 -- T_121501391__Komló_alállomás/LConn3 -- Komló_–_Sikonda_CN_235409083_120000_CN_121501391_120000/LConn3 -- bus75/LConn1
  T_336632820__Szekszárd_alállomás/LConn1 -- Pécsi_Hőerőmű–(Bonyhád_–_Szekszárd_–_Paks)_Komló_CN_302192173_120000_CN_336632820_120000/RConn1
  T_336632820__Szekszárd_alállomás/LConn2 -- Pécsi_Hőerőmű–(Bonyhád_–_Szekszárd_–_Paks)_Komló_CN_302192173_120000_CN_336632820_120000/RConn2
  Pécsi_Hőerőmű–(Bonyhád_–_Szekszárd_–_Paks)_Komló_CN_302192173_120000_CN_336632820_120000/RConn3 -- T_336632820__Szekszárd_alállomás/LConn3 -- bus76/LConn1
  Pécsi_Hőerőmű–(Bonyhád_–_Szekszárd_–_Paks)_Komló_CN_302192173_120000_CN_100788162_120000/RConn1 -- T_100788162__Paks_alállomás/RConn1 -- _CN_104062252_120000_CN_100788162_120000/LConn1 -- _CN_100788162_120000_CN_110144980_120000/LConn1 -- L_100788162/LConn1
  Pécsi_Hőerőmű–(Bonyhád_–_Szekszárd_–_Paks)_Komló_CN_302192173_120000_CN_100788162_120000/RConn2 -- T_100788162__Paks_alállomás/RConn2 -- _CN_104062252_120000_CN_100788162_120000/LConn2 -- _CN_100788162_120000_CN_110144980_120000/LConn2 -- L_100788162/LConn2
  Pécsi_Hőerőmű–(Bonyhád_–_Szekszárd_–_Paks)_Komló_CN_302192173_120000_CN_100788162_120000/RConn3 -- T_100788162__Paks_alállomás/RConn3 -- _CN_104062252_120000_CN_100788162_120000/LConn3 -- _CN_100788162_120000_CN_110144980_120000/LConn3 -- L_100788162/LConn3 -- bus77/LConn1
  T_331140850__Pécs_Kelet_alállomás/LConn1 -- Pécsi_Hőerőmű_–_Komló_CN_302192173_120000_CN_331140850_120000/RConn1
  T_331140850__Pécs_Kelet_alállomás/LConn2 -- Pécsi_Hőerőmű_–_Komló_CN_302192173_120000_CN_331140850_120000/RConn2
  Pécsi_Hőerőmű_–_Komló_CN_302192173_120000_CN_331140850_120000/RConn3 -- T_331140850__Pécs_Kelet_alállomás/LConn3 -- bus78/LConn1
  Pécsi_Hőerőmű–Mohács_CN_302192173_120000_CN_156193065_120000/RConn1 -- T_156193065__Mohács_120_kV_alállomás/LConn1 -- Baja–Mohács_CN_156193065_120000_CN_283715413_120000/LConn1
  Pécsi_Hőerőmű–Mohács_CN_302192173_120000_CN_156193065_120000/RConn2 -- T_156193065__Mohács_120_kV_alállomás/LConn2 -- Baja–Mohács_CN_156193065_120000_CN_283715413_120000/LConn2
  Pécsi_Hőerőmű–Mohács_CN_302192173_120000_CN_156193065_120000/RConn3 -- T_156193065__Mohács_120_kV_alállomás/LConn3 -- Baja–Mohács_CN_156193065_120000_CN_283715413_120000/LConn3 -- bus79/LConn1
  _CN_302192175_120000_CN_124244078_120000/LConn1 -- T_302192175__Győr_Dél_alállomás/LConn1 -- _CN_302192175_120000_CN_206353058_120000/LConn1
  _CN_302192175_120000_CN_124244078_120000/LConn2 -- T_302192175__Győr_Dél_alállomás/LConn2 -- _CN_302192175_120000_CN_206353058_120000/LConn2
  _CN_302192175_120000_CN_124244078_120000/LConn3 -- T_302192175__Győr_Dél_alállomás/LConn3 -- _CN_302192175_120000_CN_206353058_120000/LConn3 -- bus80/LConn1
  _CN_302192175_120000_CN_124244078_120000/RConn1 -- T_124244078__Győr_Kelet_alállomás/RConn1 -- _CN_124244078_120000_CN_350230665_120000/RConn1 -- _CN_124244078_120000_CN_314931464_120000/LConn1 -- Győr–Pápa_CN_124244078_120000_CN_313625037_120000/LConn1 -- L_124244078/LConn1
  _CN_302192175_120000_CN_124244078_120000/RConn2 -- T_124244078__Győr_Kelet_alállomás/RConn2 -- _CN_124244078_120000_CN_350230665_120000/RConn2 -- _CN_124244078_120000_CN_314931464_120000/LConn2 -- Győr–Pápa_CN_124244078_120000_CN_313625037_120000/LConn2 -- L_124244078/LConn2
  _CN_302192175_120000_CN_124244078_120000/RConn3 -- T_124244078__Győr_Kelet_alállomás/RConn3 -- _CN_124244078_120000_CN_350230665_120000/RConn3 -- _CN_124244078_120000_CN_314931464_120000/LConn3 -- Győr–Pápa_CN_124244078_120000_CN_313625037_120000/LConn3 -- L_124244078/LConn3 -- bus81/LConn1
  _CN_302192175_120000_CN_206353058_120000/RConn1 -- T_206353058__Károlyháza_alállomás/LConn1 -- _CN_302192176_120000_CN_206353058_120000/LConn1 -- Kapuvár___Károlyháza_CN_206353058_120000_CN_178641777_120000/LConn1 -- Kapuvár___Károlyháza_CN_206353058_120000_CN_275352278_120000/LConn1
  _CN_302192175_120000_CN_206353058_120000/RConn2 -- T_206353058__Károlyháza_alállomás/LConn2 -- _CN_302192176_120000_CN_206353058_120000/LConn2 -- Kapuvár___Károlyháza_CN_206353058_120000_CN_178641777_120000/LConn2 -- Kapuvár___Károlyháza_CN_206353058_120000_CN_275352278_120000/LConn2
  _CN_302192175_120000_CN_206353058_120000/RConn3 -- T_206353058__Károlyháza_alállomás/LConn3 -- _CN_302192176_120000_CN_206353058_120000/LConn3 -- Kapuvár___Károlyháza_CN_206353058_120000_CN_178641777_120000/LConn3 -- Kapuvár___Károlyháza_CN_206353058_120000_CN_275352278_120000/LConn3 -- bus82/LConn1
  T_302192176__Mosonmagyaróvár_alállomás/LConn1 -- _CN_302192176_120000_CN_206353058_120000/RConn1
  T_302192176__Mosonmagyaróvár_alállomás/LConn2 -- _CN_302192176_120000_CN_206353058_120000/RConn2
  _CN_302192176_120000_CN_206353058_120000/RConn3 -- T_302192176__Mosonmagyaróvár_alállomás/LConn3 -- bus83/LConn1
  Kiskundorozsma___Sándorfalva_Kiskunhalas_CN_155021873_120000_CN_100962927_120000/LConn1 -- T_155021873__Kiskundorozsma_alállomás/LConn1 -- Kiskundorozsma___Sándorfalva_Kiskunhalas_CN_155021873_120000_CN_284549184_120000/LConn1
  Kiskundorozsma___Sándorfalva_Kiskunhalas_CN_155021873_120000_CN_100962927_120000/LConn2 -- T_155021873__Kiskundorozsma_alállomás/LConn2 -- Kiskundorozsma___Sándorfalva_Kiskunhalas_CN_155021873_120000_CN_284549184_120000/LConn2
  Kiskundorozsma___Sándorfalva_Kiskunhalas_CN_155021873_120000_CN_100962927_120000/LConn3 -- T_155021873__Kiskundorozsma_alállomás/LConn3 -- Kiskundorozsma___Sándorfalva_Kiskunhalas_CN_155021873_120000_CN_284549184_120000/LConn3 -- bus84/LConn1
  Kiskundorozsma___Sándorfalva_Kiskunhalas_CN_155021873_120000_CN_100962927_120000/RConn1 -- T_100962927__Sándorfalva_alállomás/RConn4 -- _CN_398994184_120000_CN_100962927_120000/LConn1 -- Szeged___Sándorfalva_CN_100962927_120000_CN_111678830_120000/RConn1 -- Sándorfalva___Kiskunfélegyháza_CN_100962927_120000_CN_285317363_120000/RConn1 -- Sándorfalva___Kiskunfélegyháza_CN_100962927_120000_CN_370667810_120000/LConn1 -- Sándorfalva___Kiskunfélegyháza_CN_100962927_120000_CN_280595113_120000/LConn1 -- L_100962927/LConn1
  Kiskundorozsma___Sándorfalva_Kiskunhalas_CN_155021873_120000_CN_100962927_120000/RConn2 -- T_100962927__Sándorfalva_alállomás/RConn5 -- _CN_398994184_120000_CN_100962927_120000/LConn2 -- Szeged___Sándorfalva_CN_100962927_120000_CN_111678830_120000/RConn2 -- Sándorfalva___Kiskunfélegyháza_CN_100962927_120000_CN_285317363_120000/RConn2 -- Sándorfalva___Kiskunfélegyháza_CN_100962927_120000_CN_370667810_120000/LConn2 -- Sándorfalva___Kiskunfélegyháza_CN_100962927_120000_CN_280595113_120000/LConn2 -- L_100962927/LConn2
  Kiskundorozsma___Sándorfalva_Kiskunhalas_CN_155021873_120000_CN_100962927_120000/RConn3 -- T_100962927__Sándorfalva_alállomás/RConn6 -- _CN_398994184_120000_CN_100962927_120000/LConn3 -- Szeged___Sándorfalva_CN_100962927_120000_CN_111678830_120000/RConn3 -- Sándorfalva___Kiskunfélegyháza_CN_100962927_120000_CN_285317363_120000/RConn3 -- Sándorfalva___Kiskunfélegyháza_CN_100962927_120000_CN_370667810_120000/LConn3 -- Sándorfalva___Kiskunfélegyháza_CN_100962927_120000_CN_280595113_120000/LConn3 -- L_100962927/LConn3 -- bus85/LConn1
  Kiskundorozsma___Sándorfalva_Kiskunhalas_CN_155021873_120000_CN_284549184_120000/RConn1 -- T_284549184__Kiskunhalas/LConn1 -- _CN_283715413_120000_CN_284549184_120000/LConn1
  Kiskundorozsma___Sándorfalva_Kiskunhalas_CN_155021873_120000_CN_284549184_120000/RConn2 -- T_284549184__Kiskunhalas/LConn2 -- _CN_283715413_120000_CN_284549184_120000/LConn2
  Kiskundorozsma___Sándorfalva_Kiskunhalas_CN_155021873_120000_CN_284549184_120000/RConn3 -- T_284549184__Kiskunhalas/LConn3 -- _CN_283715413_120000_CN_284549184_120000/LConn3 -- bus86/LConn1
  _CN_167896114_120000_CN_296112525_120000/LConn1 -- T_167896114__/RConn1 -- _CN_167896114_120000_CN_354875849_120000/LConn1 -- _CN_167896114_120000_CN_304275625_120000/LConn1 -- L_167896114/LConn1 -- _CN_167896114_120000_CN_155803703_120000/LConn1 -- _CN_167896114_120000_CN_296944282_120000/LConn1
  _CN_167896114_120000_CN_296112525_120000/LConn2 -- T_167896114__/RConn2 -- _CN_167896114_120000_CN_354875849_120000/LConn2 -- _CN_167896114_120000_CN_304275625_120000/LConn2 -- L_167896114/LConn2 -- _CN_167896114_120000_CN_155803703_120000/LConn2 -- _CN_167896114_120000_CN_296944282_120000/LConn2
  _CN_167896114_120000_CN_296112525_120000/LConn3 -- T_167896114__/RConn3 -- _CN_167896114_120000_CN_354875849_120000/LConn3 -- _CN_167896114_120000_CN_304275625_120000/LConn3 -- L_167896114/LConn3 -- bus87/LConn1 -- _CN_167896114_120000_CN_155803703_120000/LConn3 -- _CN_167896114_120000_CN_296944282_120000/LConn3
  _CN_167896114_120000_CN_296112525_120000/RConn1 -- T_296112525__/LConn1 -- _CN_294895233_120000_CN_296112525_120000/LConn1
  _CN_167896114_120000_CN_296112525_120000/RConn2 -- T_296112525__/LConn2 -- _CN_294895233_120000_CN_296112525_120000/LConn2
  _CN_167896114_120000_CN_296112525_120000/RConn3 -- T_296112525__/LConn3 -- _CN_294895233_120000_CN_296112525_120000/LConn3 -- bus88/LConn1
  _CN_167896114_120000_CN_155803703_120000/RConn1 -- T_155803703__Felsőzsolca_alállomás/RConn1 -- _CN_155803703_120000_CN_284478605_120000/LConn1 -- _CN_155803703_120000_CN_155227474_120000/LConn1 -- L_155803703/LConn1 -- _CN_155803703_120000_CN_297281902_120000/LConn1
  _CN_167896114_120000_CN_155803703_120000/RConn2 -- T_155803703__Felsőzsolca_alállomás/RConn2 -- _CN_155803703_120000_CN_284478605_120000/LConn2 -- _CN_155803703_120000_CN_155227474_120000/LConn2 -- L_155803703/LConn2 -- _CN_155803703_120000_CN_297281902_120000/LConn2
  _CN_167896114_120000_CN_155803703_120000/RConn3 -- T_155803703__Felsőzsolca_alállomás/RConn3 -- _CN_155803703_120000_CN_284478605_120000/LConn3 -- _CN_155803703_120000_CN_155227474_120000/LConn3 -- L_155803703/LConn3 -- bus89/LConn1 -- _CN_155803703_120000_CN_297281902_120000/LConn3
  T_296944282__/LConn1 -- _CN_167896114_120000_CN_296944282_120000/RConn1
  T_296944282__/LConn2 -- _CN_167896114_120000_CN_296944282_120000/RConn2
  _CN_167896114_120000_CN_296944282_120000/RConn3 -- T_296944282__/LConn3 -- bus90/LConn1
  _CN_167896114_120000_CN_354875849_120000/RConn1 -- T_354875849__/LConn1 -- _CN_302147975_120000_CN_354875849_120000/LConn1
  _CN_167896114_120000_CN_354875849_120000/RConn2 -- T_354875849__/LConn2 -- _CN_302147975_120000_CN_354875849_120000/LConn2
  _CN_167896114_120000_CN_354875849_120000/RConn3 -- T_354875849__/LConn3 -- _CN_302147975_120000_CN_354875849_120000/LConn3 -- bus91/LConn1
  T_304275625__/LConn1 -- _CN_167896114_120000_CN_304275625_120000/RConn1
  T_304275625__/LConn2 -- _CN_167896114_120000_CN_304275625_120000/RConn2
  _CN_167896114_120000_CN_304275625_120000/RConn3 -- T_304275625__/LConn3 -- bus92/LConn1
  Nádudvar___Püspökladány_Debrecen_CN_285825715_120000_CN_256857667_120000/LConn1 -- T_285825715_120000;20000_Nádudvar_120_20_kV_alállomás/LConn1 -- Nádudvar___Püspökladány_Debrecen_CN_285825715_120000_CN_204662161_120000/LConn1 -- Nádudvar___Püspökladány_Debrecen_CN_285825715_120000_CN_251018027_120000/LConn1
  Nádudvar___Püspökladány_Debrecen_CN_285825715_120000_CN_256857667_120000/LConn2 -- T_285825715_120000;20000_Nádudvar_120_20_kV_alállomás/LConn2 -- Nádudvar___Püspökladány_Debrecen_CN_285825715_120000_CN_204662161_120000/LConn2 -- Nádudvar___Püspökladány_Debrecen_CN_285825715_120000_CN_251018027_120000/LConn2
  Nádudvar___Püspökladány_Debrecen_CN_285825715_120000_CN_256857667_120000/LConn3 -- T_285825715_120000;20000_Nádudvar_120_20_kV_alállomás/LConn3 -- Nádudvar___Püspökladány_Debrecen_CN_285825715_120000_CN_204662161_120000/LConn3 -- Nádudvar___Püspökladány_Debrecen_CN_285825715_120000_CN_251018027_120000/LConn3 -- bus93/LConn1
  T_256857667__Püspökladány_120_kV_alállomás/LConn1 -- Nádudvar___Püspökladány_Debrecen_CN_285825715_120000_CN_256857667_120000/RConn1
  T_256857667__Püspökladány_120_kV_alállomás/LConn2 -- Nádudvar___Püspökladány_Debrecen_CN_285825715_120000_CN_256857667_120000/RConn2
  Nádudvar___Püspökladány_Debrecen_CN_285825715_120000_CN_256857667_120000/RConn3 -- T_256857667__Püspökladány_120_kV_alállomás/LConn3 -- bus94/LConn1
  Nádudvar___Püspökladány_Debrecen_CN_285825715_120000_CN_204662161_120000/RConn1 -- T_204662161_120000;20000_Berettyóújfalu_120_20_kV_alállomás/LConn1 -- Debrecen___Berettyóújfalu_CN_104033901_120000_CN_204662161_120000/LConn1
  Nádudvar___Püspökladány_Debrecen_CN_285825715_120000_CN_204662161_120000/RConn2 -- T_204662161_120000;20000_Berettyóújfalu_120_20_kV_alállomás/LConn2 -- Debrecen___Berettyóújfalu_CN_104033901_120000_CN_204662161_120000/LConn2
  Nádudvar___Püspökladány_Debrecen_CN_285825715_120000_CN_204662161_120000/RConn3 -- T_204662161_120000;20000_Berettyóújfalu_120_20_kV_alállomás/LConn3 -- Debrecen___Berettyóújfalu_CN_104033901_120000_CN_204662161_120000/LConn3 -- bus95/LConn1
  Nádudvar___Püspökladány_Debrecen_CN_285825715_120000_CN_251018027_120000/RConn1 -- T_251018027_220000;120000_Tiszalök_220_120_kV_alállomás/LConn1 -- Tiszalök_Nyíregyháza_CN_292353077_120000_CN_251018027_120000/RConn1 -- _CN_251018027_120000_CN_289183615_120000/RConn1
  Nádudvar___Püspökladány_Debrecen_CN_285825715_120000_CN_251018027_120000/RConn2 -- T_251018027_220000;120000_Tiszalök_220_120_kV_alállomás/LConn2 -- Tiszalök_Nyíregyháza_CN_292353077_120000_CN_251018027_120000/RConn2 -- _CN_251018027_120000_CN_289183615_120000/RConn2
  Nádudvar___Püspökladány_Debrecen_CN_285825715_120000_CN_251018027_120000/RConn3 -- T_251018027_220000;120000_Tiszalök_220_120_kV_alállomás/LConn3 -- Tiszalök_Nyíregyháza_CN_292353077_120000_CN_251018027_120000/RConn3 -- _CN_251018027_120000_CN_289183615_120000/RConn3 -- bus96/LConn1
  Kisvárda_–_Nyíregyháza_CN_292353077_120000_CN_289912792_120000/RConn1 -- T_289912792__Kisvárda/RConn1 -- _CN_290158092_120000_CN_289912792_120000/LConn1 -- Károlyfalva–Kisvárda_120_kV_CN_289912792_120000_CN_281860578_120000/LConn1 -- L_289912792/LConn1
  Kisvárda_–_Nyíregyháza_CN_292353077_120000_CN_289912792_120000/RConn2 -- T_289912792__Kisvárda/RConn2 -- _CN_290158092_120000_CN_289912792_120000/LConn2 -- Károlyfalva–Kisvárda_120_kV_CN_289912792_120000_CN_281860578_120000/LConn2 -- L_289912792/LConn2
  Kisvárda_–_Nyíregyháza_CN_292353077_120000_CN_289912792_120000/RConn3 -- T_289912792__Kisvárda/RConn3 -- _CN_290158092_120000_CN_289912792_120000/LConn3 -- Károlyfalva–Kisvárda_120_kV_CN_289912792_120000_CN_281860578_120000/LConn3 -- L_289912792/LConn3 -- bus97/LConn1
  _CN_100863542_120000_CN_103977434_120000/RConn1 -- T_103977434__/LConn1 -- _CN_103965083_120000_CN_103977434_120000/RConn1 -- _CN_215137750_120000_CN_103977434_120000/LConn1
  _CN_100863542_120000_CN_103977434_120000/RConn2 -- T_103977434__/LConn2 -- _CN_103965083_120000_CN_103977434_120000/RConn2 -- _CN_215137750_120000_CN_103977434_120000/LConn2
  _CN_100863542_120000_CN_103977434_120000/RConn3 -- T_103977434__/LConn3 -- _CN_103965083_120000_CN_103977434_120000/RConn3 -- _CN_215137750_120000_CN_103977434_120000/LConn3 -- bus98/LConn1
  T_297281902__/LConn1 -- _CN_155803703_120000_CN_297281902_120000/RConn1
  T_297281902__/LConn2 -- _CN_155803703_120000_CN_297281902_120000/RConn2
  _CN_155803703_120000_CN_297281902_120000/RConn3 -- T_297281902__/LConn3 -- bus99/LConn1
  T_284478605__/LConn1 -- _CN_155803703_120000_CN_284478605_120000/RConn1
  T_284478605__/LConn2 -- _CN_155803703_120000_CN_284478605_120000/RConn2
  _CN_155803703_120000_CN_284478605_120000/RConn3 -- T_284478605__/LConn3 -- bus100/LConn1
  _CN_155803703_120000_CN_155227474_120000/RConn1 -- T_155227474__Sajószöged_alállomás/RConn4 -- L_155227474/LConn1
  _CN_155803703_120000_CN_155227474_120000/RConn2 -- T_155227474__Sajószöged_alállomás/RConn5 -- L_155227474/LConn2
  _CN_155803703_120000_CN_155227474_120000/RConn3 -- T_155227474__Sajószöged_alállomás/RConn6 -- L_155227474/LConn3 -- bus101/LConn1
  _CN_288864314_120000_CN_289011848_120000/LConn1 -- T_288864314__/LConn1 -- _CN_288864314_120000_CN_288863087_120000/RConn1
  _CN_288864314_120000_CN_289011848_120000/LConn2 -- T_288864314__/LConn2 -- _CN_288864314_120000_CN_288863087_120000/RConn2
  _CN_288864314_120000_CN_289011848_120000/LConn3 -- T_288864314__/LConn3 -- _CN_288864314_120000_CN_288863087_120000/RConn3 -- bus102/LConn1
  _CN_288864314_120000_CN_289011848_120000/RConn1 -- T_289011848__/LConn1 -- _CN_252028146_120000_CN_289011848_120000/RConn1
  _CN_288864314_120000_CN_289011848_120000/RConn2 -- T_289011848__/LConn2 -- _CN_252028146_120000_CN_289011848_120000/RConn2
  _CN_288864314_120000_CN_289011848_120000/RConn3 -- T_289011848__/LConn3 -- _CN_252028146_120000_CN_289011848_120000/RConn3 -- bus103/LConn1
  _CN_104027708_120000_CN_103965083_120000/RConn1 -- T_104027708__Gödöllő_alállomás/LConn1 -- _CN_104027708_120000_CN_301002581_120000/RConn1
  _CN_104027708_120000_CN_103965083_120000/RConn2 -- T_104027708__Gödöllő_alállomás/LConn2 -- _CN_104027708_120000_CN_301002581_120000/RConn2
  _CN_104027708_120000_CN_103965083_120000/RConn3 -- T_104027708__Gödöllő_alállomás/LConn3 -- _CN_104027708_120000_CN_301002581_120000/RConn3 -- bus104/LConn1
  Balatonboglár–Balatonföldvár_CN_311788819_120000_CN_311788820_120000/LConn1 -- T_311788819__Siófok_alállomás/LConn1 -- _CN_311788819_120000_CN_31538924_120000/RConn1 -- _CN_311788819_120000_CN_272940764_120000/LConn1
  Balatonboglár–Balatonföldvár_CN_311788819_120000_CN_311788820_120000/LConn2 -- T_311788819__Siófok_alállomás/LConn2 -- _CN_311788819_120000_CN_31538924_120000/RConn2 -- _CN_311788819_120000_CN_272940764_120000/LConn2
  Balatonboglár–Balatonföldvár_CN_311788819_120000_CN_311788820_120000/LConn3 -- T_311788819__Siófok_alállomás/LConn3 -- _CN_311788819_120000_CN_31538924_120000/RConn3 -- _CN_311788819_120000_CN_272940764_120000/LConn3 -- bus105/LConn1
  Balatonboglár–Balatonföldvár_CN_311788819_120000_CN_311788820_120000/RConn1 -- T_311788820__Szőlőskislak_alállomás/LConn1 -- Keszthely___Marcali_CN_243983151_120000_CN_311788820_120000/RConn1
  Balatonboglár–Balatonföldvár_CN_311788819_120000_CN_311788820_120000/RConn2 -- T_311788820__Szőlőskislak_alállomás/LConn2 -- Keszthely___Marcali_CN_243983151_120000_CN_311788820_120000/RConn2
  Balatonboglár–Balatonföldvár_CN_311788819_120000_CN_311788820_120000/RConn3 -- T_311788820__Szőlőskislak_alállomás/LConn3 -- Keszthely___Marcali_CN_243983151_120000_CN_311788820_120000/RConn3 -- bus106/LConn1
  _CN_311788819_120000_CN_272940764_120000/RConn1 -- T_272940764__/LConn1 -- _CN_350948497_120000_CN_272940764_120000/LConn1 -- Inota_Erőmű___Litér_CN_272940764_120000_CN_65034002_120000/RConn1 -- Inotai_Erőmű–Dunamenti_Erőmű_(Százhalombatta)_CN_272940764_120000_CN_302259884_120000/LConn1 -- Inotai_Erőmű–Dunamenti_Erőmű_(Százhalombatta)_CN_272940764_120000_CN_214279016_120000/LConn1
  _CN_311788819_120000_CN_272940764_120000/RConn2 -- T_272940764__/LConn2 -- _CN_350948497_120000_CN_272940764_120000/LConn2 -- Inota_Erőmű___Litér_CN_272940764_120000_CN_65034002_120000/RConn2 -- Inotai_Erőmű–Dunamenti_Erőmű_(Százhalombatta)_CN_272940764_120000_CN_302259884_120000/LConn2 -- Inotai_Erőmű–Dunamenti_Erőmű_(Százhalombatta)_CN_272940764_120000_CN_214279016_120000/LConn2
  _CN_311788819_120000_CN_272940764_120000/RConn3 -- T_272940764__/LConn3 -- _CN_350948497_120000_CN_272940764_120000/LConn3 -- Inota_Erőmű___Litér_CN_272940764_120000_CN_65034002_120000/RConn3 -- Inotai_Erőmű–Dunamenti_Erőmű_(Százhalombatta)_CN_272940764_120000_CN_302259884_120000/LConn3 -- Inotai_Erőmű–Dunamenti_Erőmű_(Százhalombatta)_CN_272940764_120000_CN_214279016_120000/LConn3 -- bus107/LConn1
  Lenti___Nedeljanec_CN_239120448_120000_CN_243816689_120000/LConn1 -- T_239120448__Lenti_alállomás/LConn1 -- Lenti___Szentgotthárd_CN_239120448_120000_CN_303049651_120000/LConn1 -- Lenti___Szentgotthárd_CN_239120448_120000_CN_244527955_120000/LConn1
  Lenti___Nedeljanec_CN_239120448_120000_CN_243816689_120000/LConn2 -- T_239120448__Lenti_alállomás/LConn2 -- Lenti___Szentgotthárd_CN_239120448_120000_CN_303049651_120000/LConn2 -- Lenti___Szentgotthárd_CN_239120448_120000_CN_244527955_120000/LConn2
  Lenti___Nedeljanec_CN_239120448_120000_CN_243816689_120000/LConn3 -- T_239120448__Lenti_alállomás/LConn3 -- Lenti___Szentgotthárd_CN_239120448_120000_CN_303049651_120000/LConn3 -- Lenti___Szentgotthárd_CN_239120448_120000_CN_244527955_120000/LConn3 -- bus108/LConn1
  Lenti___Nedeljanec_CN_239120448_120000_CN_243816689_120000/RConn1 -- T_243816689__Söjtör_alállomás/LConn1 -- Söjtör___Keszthely_CN_243983151_120000_CN_243816689_120000/RConn1
  Lenti___Nedeljanec_CN_239120448_120000_CN_243816689_120000/RConn2 -- T_243816689__Söjtör_alállomás/LConn2 -- Söjtör___Keszthely_CN_243983151_120000_CN_243816689_120000/RConn2
  Lenti___Nedeljanec_CN_239120448_120000_CN_243816689_120000/RConn3 -- T_243816689__Söjtör_alállomás/LConn3 -- Söjtör___Keszthely_CN_243983151_120000_CN_243816689_120000/RConn3 -- bus109/LConn1
  T_303049651__Szentgotthárd_alállomás/LConn1 -- Lenti___Szentgotthárd_CN_239120448_120000_CN_303049651_120000/RConn1
  T_303049651__Szentgotthárd_alállomás/LConn2 -- Lenti___Szentgotthárd_CN_239120448_120000_CN_303049651_120000/RConn2
  Lenti___Szentgotthárd_CN_239120448_120000_CN_303049651_120000/RConn3 -- T_303049651__Szentgotthárd_alállomás/LConn3 -- bus110/LConn1
  T_244527955__Pankasz_alállomás/LConn1 -- Lenti___Szentgotthárd_CN_239120448_120000_CN_244527955_120000/RConn1
  T_244527955__Pankasz_alállomás/LConn2 -- Lenti___Szentgotthárd_CN_239120448_120000_CN_244527955_120000/RConn2
  Lenti___Szentgotthárd_CN_239120448_120000_CN_244527955_120000/RConn3 -- T_244527955__Pankasz_alállomás/LConn3 -- bus111/LConn1
  T_156269125__/LConn1 -- Dunamenti___Százhalombatta_finomító_CN_156269125_120000_CN_228355796_120000/LConn1
  T_156269125__/LConn2 -- Dunamenti___Százhalombatta_finomító_CN_156269125_120000_CN_228355796_120000/LConn2
  Dunamenti___Százhalombatta_finomító_CN_156269125_120000_CN_228355796_120000/LConn3 -- T_156269125__/LConn3 -- bus112/LConn1
  Dunamenti___Százhalombatta_finomító_CN_156269125_120000_CN_228355796_120000/RConn1 -- G_228355796_/RConn1 -- _CN_100804921_220000_CN_228355796_120000/LConn1 -- Dunamenti___Ócsa_II__CN_100844170_220000_CN_228355796_120000/LConn1 -- Dunamenti___Százhalombatta_finomító_CN_100804921_120000_CN_228355796_120000/LConn1 -- _CN_172048867_132000_CN_228355796_120000/LConn1 -- Dunamenti___Érd___Diósd___Albertfalva_CN_100804921_132000_CN_228355796_120000/LConn1 -- _CN_244038276_220000_CN_228355796_120000/LConn1 -- _CN_100851012_220000_CN_228355796_120000/LConn1 -- _CN_100804905_220000_CN_228355796_120000/LConn1
  Dunamenti___Százhalombatta_finomító_CN_156269125_120000_CN_228355796_120000/RConn2 -- G_228355796_/RConn2 -- _CN_100804921_220000_CN_228355796_120000/LConn2 -- Dunamenti___Ócsa_II__CN_100844170_220000_CN_228355796_120000/LConn2 -- Dunamenti___Százhalombatta_finomító_CN_100804921_120000_CN_228355796_120000/LConn2 -- _CN_172048867_132000_CN_228355796_120000/LConn2 -- Dunamenti___Érd___Diósd___Albertfalva_CN_100804921_132000_CN_228355796_120000/LConn2 -- _CN_244038276_220000_CN_228355796_120000/LConn2 -- _CN_100851012_220000_CN_228355796_120000/LConn2 -- _CN_100804905_220000_CN_228355796_120000/LConn2
  Dunamenti___Százhalombatta_finomító_CN_156269125_120000_CN_228355796_120000/RConn3 -- G_228355796_/RConn3 -- _CN_100804921_220000_CN_228355796_120000/LConn3 -- bus113/LConn1 -- Dunamenti___Ócsa_II__CN_100844170_220000_CN_228355796_120000/LConn3 -- Dunamenti___Százhalombatta_finomító_CN_100804921_120000_CN_228355796_120000/LConn3 -- _CN_172048867_132000_CN_228355796_120000/LConn3 -- Dunamenti___Érd___Diósd___Albertfalva_CN_100804921_132000_CN_228355796_120000/LConn3 -- _CN_244038276_220000_CN_228355796_120000/LConn3 -- _CN_100851012_220000_CN_228355796_120000/LConn3 -- _CN_100804905_220000_CN_228355796_120000/LConn3
  T_267155016__Győr_Nádorváros_alállomás/LConn1 -- _CN_267155016_120000_CN_350230665_120000/RConn1
  T_267155016__Győr_Nádorváros_alállomás/LConn2 -- _CN_267155016_120000_CN_350230665_120000/RConn2
  _CN_267155016_120000_CN_350230665_120000/RConn3 -- T_267155016__Győr_Nádorváros_alállomás/LConn3 -- bus114/LConn1
  T_290158092__/LConn1 -- _CN_290158092_120000_CN_289912792_120000/RConn1
  T_290158092__/LConn2 -- _CN_290158092_120000_CN_289912792_120000/RConn2
  _CN_290158092_120000_CN_289912792_120000/RConn3 -- T_290158092__/LConn3 -- bus115/LConn1
  _CN_311977547_120000_CN_311977556_120000/LConn1 -- T_311977547__/LConn1 -- _CN_311977547_120000_CN_301495268_120000/LConn1
  _CN_311977547_120000_CN_311977556_120000/LConn2 -- T_311977547__/LConn2 -- _CN_311977547_120000_CN_301495268_120000/LConn2
  _CN_311977547_120000_CN_311977556_120000/LConn3 -- T_311977547__/LConn3 -- _CN_311977547_120000_CN_301495268_120000/LConn3 -- bus116/LConn1
  T_311977556__/LConn1 -- _CN_311977547_120000_CN_311977556_120000/RConn1
  T_311977556__/LConn2 -- _CN_311977547_120000_CN_311977556_120000/RConn2
  _CN_311977547_120000_CN_311977556_120000/RConn3 -- T_311977556__/LConn3 -- bus117/LConn1
  T_301495268__Kisigmánd_szélerőmű_alállomás/LConn1 -- _CN_311977547_120000_CN_301495268_120000/RConn1
  T_301495268__Kisigmánd_szélerőmű_alállomás/LConn2 -- _CN_311977547_120000_CN_301495268_120000/RConn2
  _CN_311977547_120000_CN_301495268_120000/RConn3 -- T_301495268__Kisigmánd_szélerőmű_alállomás/LConn3 -- bus118/LConn1
  T_248973389__/LConn1 -- _CN_248973389_120000_CN_203076074_120000/LConn1
  T_248973389__/LConn2 -- _CN_248973389_120000_CN_203076074_120000/LConn2
  _CN_248973389_120000_CN_203076074_120000/LConn3 -- T_248973389__/LConn3 -- bus119/LConn1
  T_203076074__Felsőbabád_alállomás/LConn1 -- _CN_248973389_120000_CN_203076074_120000/RConn1
  T_203076074__Felsőbabád_alállomás/LConn2 -- _CN_248973389_120000_CN_203076074_120000/RConn2
  _CN_248973389_120000_CN_203076074_120000/RConn3 -- T_203076074__Felsőbabád_alállomás/LConn3 -- bus120/LConn1
  T_398994184__/LConn1 -- _CN_398994184_120000_CN_100962927_120000/RConn1
  T_398994184__/LConn2 -- _CN_398994184_120000_CN_100962927_120000/RConn2
  _CN_398994184_120000_CN_100962927_120000/RConn3 -- T_398994184__/LConn3 -- bus121/LConn1
  T_315669517__MÁV_Kaposfüred_alállomás/LConn1 -- Kaposvár–Kaposfüred_CN_315669517_120000_CN_31538924_120000/RConn1
  T_315669517__MÁV_Kaposfüred_alállomás/LConn2 -- Kaposvár–Kaposfüred_CN_315669517_120000_CN_31538924_120000/RConn2
  Kaposvár–Kaposfüred_CN_315669517_120000_CN_31538924_120000/RConn3 -- T_315669517__MÁV_Kaposfüred_alállomás/LConn3 -- bus122/LConn1
  T_253313106_120000_/LConn1 -- _CN_253313106_120000_CN_253313109_120000/LConn1
  T_253313106_120000_/LConn2 -- _CN_253313106_120000_CN_253313109_120000/LConn2
  _CN_253313106_120000_CN_253313109_120000/LConn3 -- T_253313106_120000_/LConn3 -- bus123/LConn1
  _CN_253313106_120000_CN_253313109_120000/RConn1 -- T_253313109_120000_/LConn1 -- _CN_253313109_120000_CN_253272731_120000/LConn1 -- _CN_253313109_120000_CN_100872886_120000/RConn1
  _CN_253313106_120000_CN_253313109_120000/RConn2 -- T_253313109_120000_/LConn2 -- _CN_253313109_120000_CN_253272731_120000/LConn2 -- _CN_253313109_120000_CN_100872886_120000/RConn2
  _CN_253313106_120000_CN_253313109_120000/RConn3 -- T_253313109_120000_/LConn3 -- _CN_253313109_120000_CN_253272731_120000/LConn3 -- bus124/LConn1 -- _CN_253313109_120000_CN_100872886_120000/RConn3
  T_253272731_120000_/LConn1 -- _CN_253313109_120000_CN_253272731_120000/RConn1
  T_253272731_120000_/LConn2 -- _CN_253313109_120000_CN_253272731_120000/RConn2
  _CN_253313109_120000_CN_253272731_120000/RConn3 -- T_253272731_120000_/LConn3 -- bus125/LConn1
  Lábatlan___Tata_Dorog_CN_281841238_120000_CN_254916093_120000/LConn1 -- T_281841238__Lábatlan_alállomás/LConn1 -- Lábatlan___Tata_Dorog_CN_281841238_120000_CN_209157413_120000/LConn1
  Lábatlan___Tata_Dorog_CN_281841238_120000_CN_254916093_120000/LConn2 -- T_281841238__Lábatlan_alállomás/LConn2 -- Lábatlan___Tata_Dorog_CN_281841238_120000_CN_209157413_120000/LConn2
  Lábatlan___Tata_Dorog_CN_281841238_120000_CN_254916093_120000/LConn3 -- T_281841238__Lábatlan_alállomás/LConn3 -- Lábatlan___Tata_Dorog_CN_281841238_120000_CN_209157413_120000/LConn3 -- bus126/LConn1
  T_254916093__Tata_alállomás/LConn1 -- Lábatlan___Tata_Dorog_CN_281841238_120000_CN_254916093_120000/RConn1
  T_254916093__Tata_alállomás/LConn2 -- Lábatlan___Tata_Dorog_CN_281841238_120000_CN_254916093_120000/RConn2
  Lábatlan___Tata_Dorog_CN_281841238_120000_CN_254916093_120000/RConn3 -- T_254916093__Tata_alállomás/LConn3 -- bus127/LConn1
  Lábatlan___Tata_Dorog_CN_281841238_120000_CN_209157413_120000/RConn1 -- T_209157413_120000_Dorog_alállomás/LConn1 -- _CN_209157413_120000_CN_252727452_120000/RConn1
  Lábatlan___Tata_Dorog_CN_281841238_120000_CN_209157413_120000/RConn2 -- T_209157413_120000_Dorog_alállomás/LConn2 -- _CN_209157413_120000_CN_252727452_120000/RConn2
  Lábatlan___Tata_Dorog_CN_281841238_120000_CN_209157413_120000/RConn3 -- T_209157413_120000_Dorog_alállomás/LConn3 -- _CN_209157413_120000_CN_252727452_120000/RConn3 -- bus128/LConn1
  T_204596172_120000_Szombathely_Szőlős_alállomás/LConn1 -- _CN_245836377_120000_CN_204596172_120000/RConn1
  T_204596172_120000_Szombathely_Szőlős_alállomás/LConn2 -- _CN_245836377_120000_CN_204596172_120000/RConn2
  _CN_245836377_120000_CN_204596172_120000/RConn3 -- T_204596172_120000_Szombathely_Szőlős_alállomás/LConn3 -- bus129/LConn1
  _CN_245836377_120000_CN_166155511_120000/RConn1 -- T_166155511_400000;120000_Szombathely_400_120_kV_alállomás/RConn1 -- L_166155511/LConn1
  _CN_245836377_120000_CN_166155511_120000/RConn2 -- T_166155511_400000;120000_Szombathely_400_120_kV_alállomás/RConn2 -- L_166155511/LConn2
  _CN_245836377_120000_CN_166155511_120000/RConn3 -- T_166155511_400000;120000_Szombathely_400_120_kV_alállomás/RConn3 -- L_166155511/LConn3 -- bus130/LConn1
  _CN_245836377_120000_CN_178641777_120000/RConn1 -- T_178641777_120000;35000;20000_Sopronkövesd_E_ON_ÉDÁSZ_120_35_20_kV_alállomás/LConn1 -- Kapuvár___Károlyháza_CN_206353058_120000_CN_178641777_120000/RConn1 -- _CN_312136451_120000_CN_178641777_120000/LConn1
  _CN_245836377_120000_CN_178641777_120000/RConn2 -- T_178641777_120000;35000;20000_Sopronkövesd_E_ON_ÉDÁSZ_120_35_20_kV_alállomás/LConn2 -- Kapuvár___Károlyháza_CN_206353058_120000_CN_178641777_120000/RConn2 -- _CN_312136451_120000_CN_178641777_120000/LConn2
  _CN_245836377_120000_CN_178641777_120000/RConn3 -- T_178641777_120000;35000;20000_Sopronkövesd_E_ON_ÉDÁSZ_120_35_20_kV_alállomás/LConn3 -- Kapuvár___Károlyháza_CN_206353058_120000_CN_178641777_120000/RConn3 -- _CN_312136451_120000_CN_178641777_120000/LConn3 -- bus131/LConn1
  _CN_245836377_120000_CN_312831631_120000/RConn1 -- T_312831631__Körmend_alállomás/LConn1 -- _CN_312831631_120000_CN_209328058_120000/RConn1
  _CN_245836377_120000_CN_312831631_120000/RConn2 -- T_312831631__Körmend_alállomás/LConn2 -- _CN_312831631_120000_CN_209328058_120000/RConn2
  _CN_245836377_120000_CN_312831631_120000/RConn3 -- T_312831631__Körmend_alállomás/LConn3 -- _CN_312831631_120000_CN_209328058_120000/RConn3 -- bus132/LConn1
  T_287791196__/LConn1 -- _CN_287791196_120000_CN_113717515_120000/LConn1
  T_287791196__/LConn2 -- _CN_287791196_120000_CN_113717515_120000/LConn2
  _CN_287791196_120000_CN_113717515_120000/LConn3 -- T_287791196__/LConn3 -- bus133/LConn1
  _CN_287791196_120000_CN_113717515_120000/RConn1 -- T_113717515__Békéscsaba_120_kV_alállomás/LConn1 -- _CN_287647848_120000_CN_113717515_120000/LConn1 -- _CN_288254104_120000_CN_113717515_120000/LConn1 -- _CN_195168461_120000_CN_113717515_120000/LConn1
  _CN_287791196_120000_CN_113717515_120000/RConn2 -- T_113717515__Békéscsaba_120_kV_alállomás/LConn2 -- _CN_287647848_120000_CN_113717515_120000/LConn2 -- _CN_288254104_120000_CN_113717515_120000/LConn2 -- _CN_195168461_120000_CN_113717515_120000/LConn2
  _CN_287791196_120000_CN_113717515_120000/RConn3 -- T_113717515__Békéscsaba_120_kV_alállomás/LConn3 -- _CN_287647848_120000_CN_113717515_120000/LConn3 -- _CN_288254104_120000_CN_113717515_120000/LConn3 -- _CN_195168461_120000_CN_113717515_120000/LConn3 -- bus134/LConn1
  T_287647848__/LConn1 -- _CN_287647848_120000_CN_113717515_120000/RConn1
  T_287647848__/LConn2 -- _CN_287647848_120000_CN_113717515_120000/RConn2
  _CN_287647848_120000_CN_113717515_120000/RConn3 -- T_287647848__/LConn3 -- bus135/LConn1
  _CN_321513575_120000_CN_282182285_120000/LConn1 -- T_321513575__Ipari_Park_alállomás/LConn1 -- _CN_321513575_120000_CN_252028146_120000/RConn1
  _CN_321513575_120000_CN_282182285_120000/LConn2 -- T_321513575__Ipari_Park_alállomás/LConn2 -- _CN_321513575_120000_CN_252028146_120000/RConn2
  _CN_321513575_120000_CN_282182285_120000/LConn3 -- T_321513575__Ipari_Park_alállomás/LConn3 -- _CN_321513575_120000_CN_252028146_120000/RConn3 -- bus136/LConn1
  T_282182285__/LConn1 -- _CN_321513575_120000_CN_282182285_120000/RConn1
  T_282182285__/LConn2 -- _CN_321513575_120000_CN_282182285_120000/RConn2
  _CN_321513575_120000_CN_282182285_120000/RConn3 -- T_282182285__/LConn3 -- bus137/LConn1
  T_234435878__Aszófő_alállomás/LConn1 -- _CN_243983151_120000_CN_234435878_120000/RConn1
  T_234435878__Aszófő_alállomás/LConn2 -- _CN_243983151_120000_CN_234435878_120000/RConn2
  _CN_243983151_120000_CN_234435878_120000/RConn3 -- T_234435878__Aszófő_alállomás/LConn3 -- bus138/LConn1
  T_170160989__Tapolca_alállomás/LConn1 -- _CN_243983151_120000_CN_170160989_120000/RConn1
  T_170160989__Tapolca_alállomás/LConn2 -- _CN_243983151_120000_CN_170160989_120000/RConn2
  _CN_243983151_120000_CN_170160989_120000/RConn3 -- T_170160989__Tapolca_alállomás/LConn3 -- bus139/LConn1
  _CN_104033901_120000_CN_117853438_120000/LConn1 -- T_104033901_220000;120000;35000;20000;10000_Debrecen_220_120_35_20_10_kV_os_Alállomás/RConn1 -- _CN_104033901_120000_CN_289599131_120000/LConn1 -- _CN_104033901_120000_CN_140066772_120000/LConn1 -- Debrecen___Berettyóújfalu_CN_104033901_120000_CN_204662161_120000/RConn1 -- L_104033901/LConn1
  _CN_104033901_120000_CN_117853438_120000/LConn2 -- T_104033901_220000;120000;35000;20000;10000_Debrecen_220_120_35_20_10_kV_os_Alállomás/RConn2 -- _CN_104033901_120000_CN_289599131_120000/LConn2 -- _CN_104033901_120000_CN_140066772_120000/LConn2 -- Debrecen___Berettyóújfalu_CN_104033901_120000_CN_204662161_120000/RConn2 -- L_104033901/LConn2
  _CN_104033901_120000_CN_117853438_120000/LConn3 -- T_104033901_220000;120000;35000;20000;10000_Debrecen_220_120_35_20_10_kV_os_Alállomás/RConn3 -- _CN_104033901_120000_CN_289599131_120000/LConn3 -- _CN_104033901_120000_CN_140066772_120000/LConn3 -- Debrecen___Berettyóújfalu_CN_104033901_120000_CN_204662161_120000/RConn3 -- L_104033901/LConn3 -- bus140/LConn1
  T_117853438__/LConn1 -- _CN_104033901_120000_CN_117853438_120000/RConn1
  T_117853438__/LConn2 -- _CN_104033901_120000_CN_117853438_120000/RConn2
  _CN_104033901_120000_CN_117853438_120000/RConn3 -- T_117853438__/LConn3 -- bus141/LConn1
  _CN_104033901_120000_CN_289599131_120000/RConn1 -- T_289599131__Mátészalka_120Kv_22Kv/RConn1 -- _CN_289599131_120000_CN_289912791_120000/LConn1 -- L_289599131/LConn1
  _CN_104033901_120000_CN_289599131_120000/RConn2 -- T_289599131__Mátészalka_120Kv_22Kv/RConn2 -- _CN_289599131_120000_CN_289912791_120000/LConn2 -- L_289599131/LConn2
  _CN_104033901_120000_CN_289599131_120000/RConn3 -- T_289599131__Mátészalka_120Kv_22Kv/RConn3 -- _CN_289599131_120000_CN_289912791_120000/LConn3 -- L_289599131/LConn3 -- bus142/LConn1
  T_140066772__/LConn1 -- _CN_104033901_120000_CN_140066772_120000/RConn1
  T_140066772__/LConn2 -- _CN_104033901_120000_CN_140066772_120000/RConn2
  _CN_104033901_120000_CN_140066772_120000/RConn3 -- T_140066772__/LConn3 -- bus143/LConn1
  T_314931464__Csorna_alállomás/LConn1 -- _CN_124244078_120000_CN_314931464_120000/RConn1
  T_314931464__Csorna_alállomás/LConn2 -- _CN_124244078_120000_CN_314931464_120000/RConn2
  _CN_124244078_120000_CN_314931464_120000/RConn3 -- T_314931464__Csorna_alállomás/LConn3 -- bus144/LConn1
  Győr–Pápa_CN_124244078_120000_CN_313625037_120000/RConn1 -- T_313625037__Pápa_alállomás/LConn1 -- Pápa–Ajka_CN_320532045_120000_CN_313625037_120000/RConn1
  Győr–Pápa_CN_124244078_120000_CN_313625037_120000/RConn2 -- T_313625037__Pápa_alállomás/LConn2 -- Pápa–Ajka_CN_320532045_120000_CN_313625037_120000/RConn2
  Győr–Pápa_CN_124244078_120000_CN_313625037_120000/RConn3 -- T_313625037__Pápa_alállomás/LConn3 -- Pápa–Ajka_CN_320532045_120000_CN_313625037_120000/RConn3 -- bus145/LConn1
  T_370667810__/LConn1 -- Sándorfalva___Kiskunfélegyháza_CN_100962927_120000_CN_370667810_120000/RConn1
  T_370667810__/LConn2 -- Sándorfalva___Kiskunfélegyháza_CN_100962927_120000_CN_370667810_120000/RConn2
  Sándorfalva___Kiskunfélegyháza_CN_100962927_120000_CN_370667810_120000/RConn3 -- T_370667810__/LConn3 -- bus146/LConn1
  Sándorfalva___Kiskunfélegyháza_CN_100962927_120000_CN_280595113_120000/RConn1 -- T_280595113__/LConn1 -- _CN_283273093_120000_CN_280595113_120000/LConn1 -- _CN_153827138_120000_CN_280595113_120000/RConn1
  Sándorfalva___Kiskunfélegyháza_CN_100962927_120000_CN_280595113_120000/RConn2 -- T_280595113__/LConn2 -- _CN_283273093_120000_CN_280595113_120000/LConn2 -- _CN_153827138_120000_CN_280595113_120000/RConn2
  Sándorfalva___Kiskunfélegyháza_CN_100962927_120000_CN_280595113_120000/RConn3 -- T_280595113__/LConn3 -- _CN_283273093_120000_CN_280595113_120000/LConn3 -- bus147/LConn1 -- _CN_153827138_120000_CN_280595113_120000/RConn3
  T_294895233__/LConn1 -- _CN_294895233_120000_CN_296112525_120000/RConn1
  T_294895233__/LConn2 -- _CN_294895233_120000_CN_296112525_120000/RConn2
  _CN_294895233_120000_CN_296112525_120000/RConn3 -- T_294895233__/LConn3 -- bus148/LConn1
  T_253119622__Tamási_alállomás/LConn1 -- Tamási___Sárbogárd_CN_253119622_120000_CN_104062255_120000/LConn1
  T_253119622__Tamási_alállomás/LConn2 -- Tamási___Sárbogárd_CN_253119622_120000_CN_104062255_120000/LConn2
  Tamási___Sárbogárd_CN_253119622_120000_CN_104062255_120000/LConn3 -- T_253119622__Tamási_alállomás/LConn3 -- bus149/LConn1
  T_104062255__Sárbogárd_alállomás/LConn1 -- Tamási___Sárbogárd_CN_253119622_120000_CN_104062255_120000/RConn1
  T_104062255__Sárbogárd_alállomás/LConn2 -- Tamási___Sárbogárd_CN_253119622_120000_CN_104062255_120000/RConn2
  Tamási___Sárbogárd_CN_253119622_120000_CN_104062255_120000/RConn3 -- T_104062255__Sárbogárd_alállomás/LConn3 -- bus150/LConn1
  T_135952041_120000_/LConn1 -- _CN_252610696_120000_CN_135952041_120000/RConn1
  T_135952041_120000_/LConn2 -- _CN_252610696_120000_CN_135952041_120000/RConn2
  _CN_252610696_120000_CN_135952041_120000/RConn3 -- T_135952041_120000_/LConn3 -- bus151/LConn1
  T_350948497__/LConn1 -- _CN_350948497_120000_CN_272940764_120000/RConn1
  T_350948497__/LConn2 -- _CN_350948497_120000_CN_272940764_120000/RConn2
  _CN_350948497_120000_CN_272940764_120000/RConn3 -- T_350948497__/LConn3 -- bus152/LConn1
  Dunamenti___Dunavarsány_CN_351270546_120000_CN_100804921_120000/RConn1 -- T_100804921__Dunamenti/RConn4 -- Dunamenti___Százhalombatta_finomító_CN_100804921_120000_CN_228355796_120000/RConn1 -- L_100804921/LConn1
  Dunamenti___Dunavarsány_CN_351270546_120000_CN_100804921_120000/RConn2 -- T_100804921__Dunamenti/RConn5 -- Dunamenti___Százhalombatta_finomító_CN_100804921_120000_CN_228355796_120000/RConn2 -- L_100804921/LConn2
  Dunamenti___Dunavarsány_CN_351270546_120000_CN_100804921_120000/RConn3 -- T_100804921__Dunamenti/RConn6 -- Dunamenti___Százhalombatta_finomító_CN_100804921_120000_CN_228355796_120000/RConn3 -- L_100804921/LConn3 -- bus153/LConn1
  T_288254104__/LConn1 -- _CN_288254104_120000_CN_113717515_120000/RConn1
  T_288254104__/LConn2 -- _CN_288254104_120000_CN_113717515_120000/RConn2
  _CN_288254104_120000_CN_113717515_120000/RConn3 -- T_288254104__/LConn3 -- bus154/LConn1
  T_234987164__/LConn1 -- _CN_234987164_120000_CN_110253534_120000/LConn1
  T_234987164__/LConn2 -- _CN_234987164_120000_CN_110253534_120000/LConn2
  _CN_234987164_120000_CN_110253534_120000/LConn3 -- T_234987164__/LConn3 -- bus155/LConn1
  T_110253534__/LConn1 -- _CN_234987164_120000_CN_110253534_120000/RConn1
  T_110253534__/LConn2 -- _CN_234987164_120000_CN_110253534_120000/RConn2
  _CN_234987164_120000_CN_110253534_120000/RConn3 -- T_110253534__/LConn3 -- bus156/LConn1
  T_275352278__Kapuvár_alállomás/LConn1 -- Kapuvár___Károlyháza_CN_206353058_120000_CN_275352278_120000/RConn1
  T_275352278__Kapuvár_alállomás/LConn2 -- Kapuvár___Károlyháza_CN_206353058_120000_CN_275352278_120000/RConn2
  Kapuvár___Károlyháza_CN_206353058_120000_CN_275352278_120000/RConn3 -- T_275352278__Kapuvár_alállomás/LConn3 -- bus157/LConn1
  Mezőtúr___Békéscsaba_CN_288863087_120000_CN_287201135_120000/RConn1 -- T_287201135__Békés_120_kV_alállomás/LConn1 -- _CN_287114424_120000_CN_287201135_120000/LConn1
  Mezőtúr___Békéscsaba_CN_288863087_120000_CN_287201135_120000/RConn2 -- T_287201135__Békés_120_kV_alállomás/LConn2 -- _CN_287114424_120000_CN_287201135_120000/LConn2
  Mezőtúr___Békéscsaba_CN_288863087_120000_CN_287201135_120000/RConn3 -- T_287201135__Békés_120_kV_alállomás/LConn3 -- _CN_287114424_120000_CN_287201135_120000/LConn3 -- bus158/LConn1
  Nagybátony___Borsodnádasd_CN_173757619_120000_CN_302147975_120000/RConn1 -- T_302147975__Borsodnádasd_alállomás/LConn1 -- Eger___Borsodnádasd_CN_128526607_120000_CN_302147975_120000/LConn1 -- _CN_302147975_120000_CN_354875849_120000/RConn1
  Nagybátony___Borsodnádasd_CN_173757619_120000_CN_302147975_120000/RConn2 -- T_302147975__Borsodnádasd_alállomás/LConn2 -- Eger___Borsodnádasd_CN_128526607_120000_CN_302147975_120000/LConn2 -- _CN_302147975_120000_CN_354875849_120000/RConn2
  Nagybátony___Borsodnádasd_CN_173757619_120000_CN_302147975_120000/RConn3 -- T_302147975__Borsodnádasd_alállomás/LConn3 -- Eger___Borsodnádasd_CN_128526607_120000_CN_302147975_120000/LConn3 -- _CN_302147975_120000_CN_354875849_120000/RConn3 -- bus159/LConn1
  Salgótarján_Öntöde_–_Nagybátony_CN_173757619_120000_CN_355349327_120000/RConn1 -- T_355349327__Öntödei_alállomás/LConn1 -- Salgótarján–Salgótarján_Öntöde_CN_299521957_120000_CN_355349327_120000/LConn1
  Salgótarján_Öntöde_–_Nagybátony_CN_173757619_120000_CN_355349327_120000/RConn2 -- T_355349327__Öntödei_alállomás/LConn2 -- Salgótarján–Salgótarján_Öntöde_CN_299521957_120000_CN_355349327_120000/LConn2
  Salgótarján_Öntöde_–_Nagybátony_CN_173757619_120000_CN_355349327_120000/RConn3 -- T_355349327__Öntödei_alállomás/LConn3 -- Salgótarján–Salgótarján_Öntöde_CN_299521957_120000_CN_355349327_120000/LConn3 -- bus160/LConn1
  T_103950678__Dunakeszi_alállomás/LConn1 -- _CN_100872886_120000_CN_103950678_120000/RConn1
  T_103950678__Dunakeszi_alállomás/LConn2 -- _CN_100872886_120000_CN_103950678_120000/RConn2
  _CN_100872886_120000_CN_103950678_120000/RConn3 -- T_103950678__Dunakeszi_alállomás/LConn3 -- bus161/LConn1
  T_103950687_120000_Fót_alállomás/LConn1 -- _CN_100872886_120000_CN_103950687_120000/RConn1
  T_103950687_120000_Fót_alállomás/LConn2 -- _CN_100872886_120000_CN_103950687_120000/RConn2
  _CN_100872886_120000_CN_103950687_120000/RConn3 -- T_103950687_120000_Fót_alállomás/LConn3 -- bus162/LConn1
  T_287114424__/LConn1 -- _CN_287114424_120000_CN_287201135_120000/RConn1
  T_287114424__/LConn2 -- _CN_287114424_120000_CN_287201135_120000/RConn2
  _CN_287114424_120000_CN_287201135_120000/RConn3 -- T_287114424__/LConn3 -- bus163/LConn1
  T_291223737__Kunszentmárton_alállomás/LConn1 -- Kunszentmárton___Szentes_CN_291223737_120000_CN_288736592_120000/LConn1
  T_291223737__Kunszentmárton_alállomás/LConn2 -- Kunszentmárton___Szentes_CN_291223737_120000_CN_288736592_120000/LConn2
  Kunszentmárton___Szentes_CN_291223737_120000_CN_288736592_120000/LConn3 -- T_291223737__Kunszentmárton_alállomás/LConn3 -- bus164/LConn1
  Kunszentmárton___Szentes_CN_291223737_120000_CN_288736592_120000/RConn1 -- T_288736592__Szentes_alállomás/LConn1 -- Szentes___Hódmezővásárhely_CN_291442885_120000_CN_288736592_120000/LConn1
  Kunszentmárton___Szentes_CN_291223737_120000_CN_288736592_120000/RConn2 -- T_288736592__Szentes_alállomás/LConn2 -- Szentes___Hódmezővásárhely_CN_291442885_120000_CN_288736592_120000/LConn2
  Kunszentmárton___Szentes_CN_291223737_120000_CN_288736592_120000/RConn3 -- T_288736592__Szentes_alállomás/LConn3 -- Szentes___Hódmezővásárhely_CN_291442885_120000_CN_288736592_120000/LConn3 -- bus165/LConn1
  Komló_–_Sikonda_CN_235409083_120000_CN_121501391_120000/RConn1 -- T_235409083__Sikonda_alállomás/LConn1 -- Kaposvár_–_Sikonda_CN_235409083_120000_CN_331463129_120000/LConn1 -- Kaposvár_–_Sikonda_CN_235409083_120000_CN_31538924_120000/RConn1
  Komló_–_Sikonda_CN_235409083_120000_CN_121501391_120000/RConn2 -- T_235409083__Sikonda_alállomás/LConn2 -- Kaposvár_–_Sikonda_CN_235409083_120000_CN_331463129_120000/LConn2 -- Kaposvár_–_Sikonda_CN_235409083_120000_CN_31538924_120000/RConn2
  Komló_–_Sikonda_CN_235409083_120000_CN_121501391_120000/RConn3 -- T_235409083__Sikonda_alállomás/LConn3 -- Kaposvár_–_Sikonda_CN_235409083_120000_CN_331463129_120000/LConn3 -- Kaposvár_–_Sikonda_CN_235409083_120000_CN_31538924_120000/RConn3 -- bus166/LConn1
  T_331463129__Mindszentgodisa_alállomás/LConn1 -- Kaposvár_–_Sikonda_CN_235409083_120000_CN_331463129_120000/RConn1
  T_331463129__Mindszentgodisa_alállomás/LConn2 -- Kaposvár_–_Sikonda_CN_235409083_120000_CN_331463129_120000/RConn2
  Kaposvár_–_Sikonda_CN_235409083_120000_CN_331463129_120000/RConn3 -- T_331463129__Mindszentgodisa_alállomás/LConn3 -- bus167/LConn1
  T_291442885__Hódmezővásárhely_alállomás/LConn1 -- Szentes___Hódmezővásárhely_CN_291442885_120000_CN_288736592_120000/RConn1
  T_291442885__Hódmezővásárhely_alállomás/LConn2 -- Szentes___Hódmezővásárhely_CN_291442885_120000_CN_288736592_120000/RConn2
  Szentes___Hódmezővásárhely_CN_291442885_120000_CN_288736592_120000/RConn3 -- T_291442885__Hódmezővásárhely_alállomás/LConn3 -- bus168/LConn1
  Cegléd–Nagykőrös_CN_223956685_120000_CN_281465215_120000/LConn1 -- T_223956685__Cegléd_alállomás/RConn1 -- Szolnok–Cegléd_CN_223956685_120000_CN_252028146_120000/RConn1 -- L_223956685/LConn1 -- Cegléd–Nagykőrös_CN_223956685_120000_CN_153827138_120000/RConn1
  Cegléd–Nagykőrös_CN_223956685_120000_CN_281465215_120000/LConn2 -- T_223956685__Cegléd_alállomás/RConn2 -- Szolnok–Cegléd_CN_223956685_120000_CN_252028146_120000/RConn2 -- L_223956685/LConn2 -- Cegléd–Nagykőrös_CN_223956685_120000_CN_153827138_120000/RConn2
  Cegléd–Nagykőrös_CN_223956685_120000_CN_281465215_120000/LConn3 -- T_223956685__Cegléd_alállomás/RConn3 -- Szolnok–Cegléd_CN_223956685_120000_CN_252028146_120000/RConn3 -- L_223956685/LConn3 -- bus169/LConn1 -- Cegléd–Nagykőrös_CN_223956685_120000_CN_153827138_120000/RConn3
  T_281465215__Nagykőrös_alállomás/LConn1 -- Cegléd–Nagykőrös_CN_223956685_120000_CN_281465215_120000/RConn1
  T_281465215__Nagykőrös_alállomás/LConn2 -- Cegléd–Nagykőrös_CN_223956685_120000_CN_281465215_120000/RConn2
  Cegléd–Nagykőrös_CN_223956685_120000_CN_281465215_120000/RConn3 -- T_281465215__Nagykőrös_alállomás/LConn3 -- bus170/LConn1
  _CN_195168461_120000_CN_113717515_120000/RConn1 -- T_195168461__/RConn1 -- L_195168461/LConn1
  _CN_195168461_120000_CN_113717515_120000/RConn2 -- T_195168461__/RConn2 -- L_195168461/LConn2
  _CN_195168461_120000_CN_113717515_120000/RConn3 -- T_195168461__/RConn3 -- L_195168461/LConn3 -- bus171/LConn1
  _CN_153098964_120000_CN_136396751_120000/RConn1 -- T_153098964__Budaörs_alállomás/LConn1 -- _CN_153098964_120000_CN_173251331_120000/LConn1 -- _CN_153098964_120000_CN_254847446_120000/RConn1
  _CN_153098964_120000_CN_136396751_120000/RConn2 -- T_153098964__Budaörs_alállomás/LConn2 -- _CN_153098964_120000_CN_173251331_120000/LConn2 -- _CN_153098964_120000_CN_254847446_120000/RConn2
  _CN_153098964_120000_CN_136396751_120000/RConn3 -- T_153098964__Budaörs_alállomás/LConn3 -- _CN_153098964_120000_CN_173251331_120000/LConn3 -- _CN_153098964_120000_CN_254847446_120000/RConn3 -- bus172/LConn1
  T_173251331_120000_Biatorbágy_alállomás/LConn1 -- _CN_153098964_120000_CN_173251331_120000/RConn1
  T_173251331_120000_Biatorbágy_alállomás/LConn2 -- _CN_153098964_120000_CN_173251331_120000/RConn2
  _CN_153098964_120000_CN_173251331_120000/RConn3 -- T_173251331_120000_Biatorbágy_alállomás/LConn3 -- bus173/LConn1
  T_302259884_120000_Szabadbattyán_alállomás/LConn1 -- Inotai_Erőmű–Dunamenti_Erőmű_(Százhalombatta)_CN_272940764_120000_CN_302259884_120000/RConn1
  T_302259884_120000_Szabadbattyán_alállomás/LConn2 -- Inotai_Erőmű–Dunamenti_Erőmű_(Százhalombatta)_CN_272940764_120000_CN_302259884_120000/RConn2
  Inotai_Erőmű–Dunamenti_Erőmű_(Százhalombatta)_CN_272940764_120000_CN_302259884_120000/RConn3 -- T_302259884_120000_Szabadbattyán_alállomás/LConn3 -- bus174/LConn1
  Inotai_Erőmű–Dunamenti_Erőmű_(Százhalombatta)_CN_272940764_120000_CN_214279016_120000/RConn1 -- T_214279016__Székesfehérvár_Észak_alállomás/LConn1 -- _CN_288721741_120000_CN_214279016_120000/LConn1
  Inotai_Erőmű–Dunamenti_Erőmű_(Százhalombatta)_CN_272940764_120000_CN_214279016_120000/RConn2 -- T_214279016__Székesfehérvár_Észak_alállomás/LConn2 -- _CN_288721741_120000_CN_214279016_120000/LConn2
  Inotai_Erőmű–Dunamenti_Erőmű_(Százhalombatta)_CN_272940764_120000_CN_214279016_120000/RConn3 -- T_214279016__Székesfehérvár_Észak_alállomás/LConn3 -- _CN_288721741_120000_CN_214279016_120000/LConn3 -- bus175/LConn1
  T_162874597__Mezőkövesd_alállomás/LConn1 -- _CN_162874597_120000_CN_235599317_120000/LConn1
  T_162874597__Mezőkövesd_alállomás/LConn2 -- _CN_162874597_120000_CN_235599317_120000/LConn2
  _CN_162874597_120000_CN_235599317_120000/LConn3 -- T_162874597__Mezőkövesd_alállomás/LConn3 -- bus176/LConn1
  _CN_162874597_120000_CN_235599317_120000/RConn1 -- T_235599317__Füzesabony_alállomás/LConn1 -- _CN_235599317_120000_CN_307229690_120000/LConn1
  _CN_162874597_120000_CN_235599317_120000/RConn2 -- T_235599317__Füzesabony_alállomás/LConn2 -- _CN_235599317_120000_CN_307229690_120000/LConn2
  _CN_162874597_120000_CN_235599317_120000/RConn3 -- T_235599317__Füzesabony_alállomás/LConn3 -- _CN_235599317_120000_CN_307229690_120000/LConn3 -- bus177/LConn1
  _CN_271034091_120000_CN_110144980_120000/LConn1 -- T_271034091__Baja_Dunapart_alállomás/LConn1 -- _CN_271034091_120000_CN_283715413_120000/LConn1
  _CN_271034091_120000_CN_110144980_120000/LConn2 -- T_271034091__Baja_Dunapart_alállomás/LConn2 -- _CN_271034091_120000_CN_283715413_120000/LConn2
  _CN_271034091_120000_CN_110144980_120000/LConn3 -- T_271034091__Baja_Dunapart_alállomás/LConn3 -- _CN_271034091_120000_CN_283715413_120000/LConn3 -- bus178/LConn1
  _CN_271034091_120000_CN_110144980_120000/RConn1 -- T_110144980__Kalocsa_120_kV_alállomás/RConn1 -- _CN_100788162_120000_CN_110144980_120000/RConn1 -- L_110144980/LConn1
  _CN_271034091_120000_CN_110144980_120000/RConn2 -- T_110144980__Kalocsa_120_kV_alállomás/RConn2 -- _CN_100788162_120000_CN_110144980_120000/RConn2 -- L_110144980/LConn2
  _CN_271034091_120000_CN_110144980_120000/RConn3 -- T_110144980__Kalocsa_120_kV_alállomás/RConn3 -- _CN_100788162_120000_CN_110144980_120000/RConn3 -- L_110144980/LConn3 -- bus179/LConn1
  _CN_271034091_120000_CN_283715413_120000/RConn1 -- T_283715413__Baja_120_kV_alállomás/LConn1 -- _CN_283715413_120000_CN_284549184_120000/RConn1 -- Baja–Mohács_CN_156193065_120000_CN_283715413_120000/RConn1
  _CN_271034091_120000_CN_283715413_120000/RConn2 -- T_283715413__Baja_120_kV_alállomás/LConn2 -- _CN_283715413_120000_CN_284549184_120000/RConn2 -- Baja–Mohács_CN_156193065_120000_CN_283715413_120000/RConn2
  _CN_271034091_120000_CN_283715413_120000/RConn3 -- T_283715413__Baja_120_kV_alállomás/LConn3 -- _CN_283715413_120000_CN_284549184_120000/RConn3 -- bus180/LConn1 -- Baja–Mohács_CN_156193065_120000_CN_283715413_120000/RConn3
  Kaposvár–Toponár_CN_31538924_120000_CN_113570302_120000/RConn1 -- T_113570302_400000;120000_Toponár_400_120_kV_alállomás/RConn1 -- L_113570302/LConn1
  Kaposvár–Toponár_CN_31538924_120000_CN_113570302_120000/RConn2 -- T_113570302_400000;120000_Toponár_400_120_kV_alállomás/RConn2 -- L_113570302/LConn2
  Kaposvár–Toponár_CN_31538924_120000_CN_113570302_120000/RConn3 -- T_113570302_400000;120000_Toponár_400_120_kV_alállomás/RConn3 -- L_113570302/LConn3 -- bus181/LConn1
  T_288863210__/LConn1 -- _CN_252028146_120000_CN_288863210_120000/RConn1
  T_288863210__/LConn2 -- _CN_252028146_120000_CN_288863210_120000/RConn2
  _CN_252028146_120000_CN_288863210_120000/RConn3 -- T_288863210__/LConn3 -- bus182/LConn1
  T_312136451__/LConn1 -- _CN_312136451_120000_CN_178641777_120000/RConn1
  T_312136451__/LConn2 -- _CN_312136451_120000_CN_178641777_120000/RConn2
  _CN_312136451_120000_CN_178641777_120000/RConn3 -- T_312136451__/LConn3 -- bus183/LConn1
  _CN_235599317_120000_CN_307229690_120000/RConn1 -- T_307229690__/LConn1 -- _CN_304280556_120000_CN_307229690_120000/LConn1
  _CN_235599317_120000_CN_307229690_120000/RConn2 -- T_307229690__/LConn2 -- _CN_304280556_120000_CN_307229690_120000/LConn2
  _CN_235599317_120000_CN_307229690_120000/RConn3 -- T_307229690__/LConn3 -- _CN_304280556_120000_CN_307229690_120000/LConn3 -- bus184/LConn1
  T_128526607__Eger_Észak_alállomás/LConn1 -- Eger___Borsodnádasd_CN_128526607_120000_CN_302147975_120000/RConn1
  T_128526607__Eger_Észak_alállomás/LConn2 -- Eger___Borsodnádasd_CN_128526607_120000_CN_302147975_120000/RConn2
  Eger___Borsodnádasd_CN_128526607_120000_CN_302147975_120000/RConn3 -- T_128526607__Eger_Észak_alállomás/LConn3 -- bus185/LConn1
  G_155044639_Litér_Tartalék_Erőmű/RConn1 -- _CN_65034002_120000_CN_155044639_120000/RConn1
  G_155044639_Litér_Tartalék_Erőmű/RConn2 -- _CN_65034002_120000_CN_155044639_120000/RConn2
  _CN_65034002_120000_CN_155044639_120000/RConn3 -- G_155044639_Litér_Tartalék_Erőmű/RConn3 -- bus186/LConn1
  T_294585306__/LConn1 -- _CN_294585306_120000_CN_294690169_120000/LConn1
  T_294585306__/LConn2 -- _CN_294585306_120000_CN_294690169_120000/LConn2
  _CN_294585306_120000_CN_294690169_120000/LConn3 -- T_294585306__/LConn3 -- bus187/LConn1
  T_294690169__Hejőcsaba_alállomás/LConn1 -- _CN_294585306_120000_CN_294690169_120000/RConn1
  T_294690169__Hejőcsaba_alállomás/LConn2 -- _CN_294585306_120000_CN_294690169_120000/RConn2
  _CN_294585306_120000_CN_294690169_120000/RConn3 -- T_294690169__Hejőcsaba_alállomás/LConn3 -- bus188/LConn1
  T_121135019_120000;20000_120_20_kV_s_Barcsi_tarnszformátor_állomás/LConn1 -- Barcs___Szigetvár_120_Kv_s_távvezeték_CN_121241890_120000_CN_121135019_120000/RConn1
  T_121135019_120000;20000_120_20_kV_s_Barcsi_tarnszformátor_állomás/LConn2 -- Barcs___Szigetvár_120_Kv_s_távvezeték_CN_121241890_120000_CN_121135019_120000/RConn2
  Barcs___Szigetvár_120_Kv_s_távvezeték_CN_121241890_120000_CN_121135019_120000/RConn3 -- T_121135019_120000;20000_120_20_kV_s_Barcsi_tarnszformátor_állomás/LConn3 -- bus189/LConn1
  T_104062252__/LConn1 -- _CN_104062252_120000_CN_100788162_120000/RConn1
  T_104062252__/LConn2 -- _CN_104062252_120000_CN_100788162_120000/RConn2
  _CN_104062252_120000_CN_100788162_120000/RConn3 -- T_104062252__/LConn3 -- bus190/LConn1
  T_283021123__Szabadszállás_alállomás/LConn1 -- _CN_153827138_120000_CN_283021123_120000/RConn1
  T_283021123__Szabadszállás_alállomás/LConn2 -- _CN_153827138_120000_CN_283021123_120000/RConn2
  _CN_153827138_120000_CN_283021123_120000/RConn3 -- T_283021123__Szabadszállás_alállomás/LConn3 -- bus191/LConn1
  Albertfalva_–_Csepel_T_–_Népliget_120_kV_CN_100851012_120000_CN_254603237_120000/LConn1 -- T_100851012_220000;12000;10000_Albertfalva_ELMŰ_132_10_kV_alállomás/RConn4 -- L_100851012/LConn1
  Albertfalva_–_Csepel_T_–_Népliget_120_kV_CN_100851012_120000_CN_254603237_120000/LConn2 -- T_100851012_220000;12000;10000_Albertfalva_ELMŰ_132_10_kV_alállomás/RConn5 -- L_100851012/LConn2
  Albertfalva_–_Csepel_T_–_Népliget_120_kV_CN_100851012_120000_CN_254603237_120000/LConn3 -- T_100851012_220000;12000;10000_Albertfalva_ELMŰ_132_10_kV_alállomás/RConn6 -- L_100851012/LConn3 -- bus192/LConn1
  Albertfalva_–_Csepel_T_–_Népliget_120_kV_CN_100851012_120000_CN_254603237_120000/RConn1 -- T_254603237_120000;10000_Népliget/LConn1 -- Népliget_CN_103965083_120000_CN_254603237_120000/RConn1
  Albertfalva_–_Csepel_T_–_Népliget_120_kV_CN_100851012_120000_CN_254603237_120000/RConn2 -- T_254603237_120000;10000_Népliget/LConn2 -- Népliget_CN_103965083_120000_CN_254603237_120000/RConn2
  Albertfalva_–_Csepel_T_–_Népliget_120_kV_CN_100851012_120000_CN_254603237_120000/RConn3 -- T_254603237_120000;10000_Népliget/LConn3 -- Népliget_CN_103965083_120000_CN_254603237_120000/RConn3 -- bus193/LConn1
  T_288721741__Dunaújváros_II__132_22_kV_os_transzformátor_állomás/LConn1 -- _CN_288721741_120000_CN_214279016_120000/RConn1
  T_288721741__Dunaújváros_II__132_22_kV_os_transzformátor_állomás/LConn2 -- _CN_288721741_120000_CN_214279016_120000/RConn2
  _CN_288721741_120000_CN_214279016_120000/RConn3 -- T_288721741__Dunaújváros_II__132_22_kV_os_transzformátor_állomás/LConn3 -- bus194/LConn1
  T_243726196_120000;11000_Kanizsavár_alállomás/LConn1 -- Kanizsavár___Nagykanizsa_CN_203404634_120000_CN_243726196_120000/RConn1
  T_243726196_120000;11000_Kanizsavár_alállomás/LConn2 -- Kanizsavár___Nagykanizsa_CN_203404634_120000_CN_243726196_120000/RConn2
  Kanizsavár___Nagykanizsa_CN_203404634_120000_CN_243726196_120000/RConn3 -- T_243726196_120000;11000_Kanizsavár_alállomás/LConn3 -- bus195/LConn1
  T_283273093__Csongrád_alállomás/LConn1 -- _CN_283273093_120000_CN_280595113_120000/RConn1
  T_283273093__Csongrád_alállomás/LConn2 -- _CN_283273093_120000_CN_280595113_120000/RConn2
  _CN_283273093_120000_CN_280595113_120000/RConn3 -- T_283273093__Csongrád_alállomás/LConn3 -- bus196/LConn1
  T_103984593__/LConn1 -- Népliget_CN_103965083_120000_CN_103984593_120000/RConn1
  T_103984593__/LConn2 -- Népliget_CN_103965083_120000_CN_103984593_120000/RConn2
  Népliget_CN_103965083_120000_CN_103984593_120000/RConn3 -- T_103984593__/LConn3 -- bus197/LConn1
  T_289912791__/LConn1 -- _CN_289599131_120000_CN_289912791_120000/RConn1
  T_289912791__/LConn2 -- _CN_289599131_120000_CN_289912791_120000/RConn2
  _CN_289599131_120000_CN_289912791_120000/RConn3 -- T_289912791__/LConn3 -- bus198/LConn1
  T_299521957__Salgótarján,_Művésztelepi_alállomás/LConn1 -- Salgótarján–Salgótarján_Öntöde_CN_299521957_120000_CN_355349327_120000/RConn1
  T_299521957__Salgótarján,_Művésztelepi_alállomás/LConn2 -- Salgótarján–Salgótarján_Öntöde_CN_299521957_120000_CN_355349327_120000/RConn2
  Salgótarján–Salgótarján_Öntöde_CN_299521957_120000_CN_355349327_120000/RConn3 -- T_299521957__Salgótarján,_Művésztelepi_alállomás/LConn3 -- bus199/LConn1
  T_215137750_120000_Rákosfalva_alállomás/LConn1 -- _CN_215137750_120000_CN_103977434_120000/RConn1
  T_215137750_120000_Rákosfalva_alállomás/LConn2 -- _CN_215137750_120000_CN_103977434_120000/RConn2
  _CN_215137750_120000_CN_103977434_120000/RConn3 -- T_215137750_120000_Rákosfalva_alállomás/LConn3 -- bus200/LConn1
  T_281860578__Károlyfalva_alállomás/LConn1 -- Károlyfalva–Kisvárda_120_kV_CN_289912792_120000_CN_281860578_120000/RConn1
  T_281860578__Károlyfalva_alállomás/LConn2 -- Károlyfalva–Kisvárda_120_kV_CN_289912792_120000_CN_281860578_120000/RConn2
  Károlyfalva–Kisvárda_120_kV_CN_289912792_120000_CN_281860578_120000/RConn3 -- T_281860578__Károlyfalva_alállomás/LConn3 -- bus201/LConn1
  T_304280556__/LConn1 -- _CN_304280556_120000_CN_307229690_120000/RConn1
  T_304280556__/LConn2 -- _CN_304280556_120000_CN_307229690_120000/RConn2
  _CN_304280556_120000_CN_307229690_120000/RConn3 -- T_304280556__/LConn3 -- bus202/LConn1
  _CN_172048867_132000_CN_100851012_132000/LConn1 -- T_172048867__ELMŰ_Rózsakert_132_10_kV_alállomás/LConn1 -- _CN_172048867_132000_CN_172049204_132000/LConn1 -- _CN_172048867_132000_CN_100848980_132000/LConn1 -- _CN_172048867_132000_CN_228355796_120000/RConn1
  _CN_172048867_132000_CN_100851012_132000/LConn2 -- T_172048867__ELMŰ_Rózsakert_132_10_kV_alállomás/LConn2 -- _CN_172048867_132000_CN_172049204_132000/LConn2 -- _CN_172048867_132000_CN_100848980_132000/LConn2 -- _CN_172048867_132000_CN_228355796_120000/RConn2
  _CN_172048867_132000_CN_100851012_132000/LConn3 -- T_172048867__ELMŰ_Rózsakert_132_10_kV_alállomás/LConn3 -- _CN_172048867_132000_CN_172049204_132000/LConn3 -- _CN_172048867_132000_CN_100848980_132000/LConn3 -- _CN_172048867_132000_CN_228355796_120000/RConn3 -- bus203/LConn1
  T_100851012_220000;12000;10000_Albertfalva_ELMŰ_132_10_kV_alállomás/RConn1 -- _CN_172048867_132000_CN_100851012_132000/RConn1
  T_100851012_220000;12000;10000_Albertfalva_ELMŰ_132_10_kV_alállomás/RConn2 -- _CN_172048867_132000_CN_100851012_132000/RConn2
  _CN_172048867_132000_CN_100851012_132000/RConn3 -- T_100851012_220000;12000;10000_Albertfalva_ELMŰ_132_10_kV_alállomás/RConn3 -- bus204/LConn1
  T_172049204__Diósd_alállomás/LConn1 -- _CN_172048867_132000_CN_172049204_132000/RConn1
  T_172049204__Diósd_alállomás/LConn2 -- _CN_172048867_132000_CN_172049204_132000/RConn2
  _CN_172048867_132000_CN_172049204_132000/RConn3 -- T_172049204__Diósd_alállomás/LConn3 -- bus205/LConn1
  T_100848980__Érd/LConn1 -- _CN_172048867_132000_CN_100848980_132000/RConn1
  T_100848980__Érd/LConn2 -- _CN_172048867_132000_CN_100848980_132000/RConn2
  _CN_172048867_132000_CN_100848980_132000/RConn3 -- T_100848980__Érd/LConn3 -- bus206/LConn1
  T_223957931__Monor_alállomás/LConn1 -- Cegléd–Monor_CN_223957931_132000_CN_223956685_132000/LConn1
  T_223957931__Monor_alállomás/LConn2 -- Cegléd–Monor_CN_223957931_132000_CN_223956685_132000/LConn2
  Cegléd–Monor_CN_223957931_132000_CN_223956685_132000/LConn3 -- T_223957931__Monor_alállomás/LConn3 -- bus207/LConn1
  T_223956685__Cegléd_alállomás/LConn1 -- Cegléd–Monor_CN_223957931_132000_CN_223956685_132000/RConn1
  T_223956685__Cegléd_alállomás/LConn2 -- Cegléd–Monor_CN_223957931_132000_CN_223956685_132000/RConn2
  Cegléd–Monor_CN_223957931_132000_CN_223956685_132000/RConn3 -- T_223956685__Cegléd_alállomás/LConn3 -- bus208/LConn1
  _CN_110144980_132000_CN_285319199_132000/LConn1 -- T_110144980__Kalocsa_120_kV_alállomás/LConn1 -- _CN_110144980_132000_CN_285581278_132000/LConn1
  _CN_110144980_132000_CN_285319199_132000/LConn2 -- T_110144980__Kalocsa_120_kV_alállomás/LConn2 -- _CN_110144980_132000_CN_285581278_132000/LConn2
  _CN_110144980_132000_CN_285319199_132000/LConn3 -- T_110144980__Kalocsa_120_kV_alállomás/LConn3 -- _CN_110144980_132000_CN_285581278_132000/LConn3 -- bus209/LConn1
  T_285319199__/LConn1 -- _CN_110144980_132000_CN_285319199_132000/RConn1
  T_285319199__/LConn2 -- _CN_110144980_132000_CN_285319199_132000/RConn2
  _CN_110144980_132000_CN_285319199_132000/RConn3 -- T_285319199__/LConn3 -- bus210/LConn1
  T_285581278__/LConn1 -- _CN_110144980_132000_CN_285581278_132000/RConn1
  T_285581278__/LConn2 -- _CN_110144980_132000_CN_285581278_132000/RConn2
  _CN_110144980_132000_CN_285581278_132000/RConn3 -- T_285581278__/LConn3 -- bus211/LConn1
  T_289912792__Kisvárda/LConn1 -- Kisvárda–Vásárosnamény–Fehérgyarmat–Mátészalka_CN_289912792_132000_CN_289599131_132000/LConn1
  T_289912792__Kisvárda/LConn2 -- Kisvárda–Vásárosnamény–Fehérgyarmat–Mátészalka_CN_289912792_132000_CN_289599131_132000/LConn2
  Kisvárda–Vásárosnamény–Fehérgyarmat–Mátészalka_CN_289912792_132000_CN_289599131_132000/LConn3 -- T_289912792__Kisvárda/LConn3 -- bus212/LConn1
  T_289599131__Mátészalka_120Kv_22Kv/LConn1 -- Kisvárda–Vásárosnamény–Fehérgyarmat–Mátészalka_CN_289912792_132000_CN_289599131_132000/RConn1
  T_289599131__Mátészalka_120Kv_22Kv/LConn2 -- Kisvárda–Vásárosnamény–Fehérgyarmat–Mátészalka_CN_289912792_132000_CN_289599131_132000/RConn2
  Kisvárda–Vásárosnamény–Fehérgyarmat–Mátészalka_CN_289912792_132000_CN_289599131_132000/RConn3 -- T_289599131__Mátészalka_120Kv_22Kv/LConn3 -- bus213/LConn1
  T_100804921__Dunamenti/RConn1 -- Dunamenti___Érd___Diósd___Albertfalva_CN_100804921_132000_CN_228355796_120000/RConn1
  T_100804921__Dunamenti/RConn2 -- Dunamenti___Érd___Diósd___Albertfalva_CN_100804921_132000_CN_228355796_120000/RConn2
  Dunamenti___Érd___Diósd___Albertfalva_CN_100804921_132000_CN_228355796_120000/RConn3 -- T_100804921__Dunamenti/RConn3 -- bus214/LConn1
  T_244038276_220000;120000_Oroszlány_alállomás/LConn1 -- _CN_244038276_220000_CN_228355796_120000/RConn1
  T_244038276_220000;120000_Oroszlány_alállomás/LConn2 -- _CN_244038276_220000_CN_228355796_120000/RConn2
  _CN_244038276_220000_CN_228355796_120000/RConn3 -- T_244038276_220000;120000_Oroszlány_alállomás/LConn3 -- bus215/LConn1
  T_100851012_220000;12000;10000_Albertfalva_ELMŰ_132_10_kV_alállomás/LConn1 -- _CN_100851012_220000_CN_228355796_120000/RConn1
  T_100851012_220000;12000;10000_Albertfalva_ELMŰ_132_10_kV_alállomás/LConn2 -- _CN_100851012_220000_CN_228355796_120000/RConn2
  _CN_100851012_220000_CN_228355796_120000/RConn3 -- T_100851012_220000;12000;10000_Albertfalva_ELMŰ_132_10_kV_alállomás/LConn3 -- bus216/LConn1
  Detk___Zugló_II__CN_100863542_220000_CN_301002581_220000/LConn1 -- T_100863542__Zugló_alállomás/LConn1 -- Göd___Zugló_CN_100863542_220000_CN_100872886_220000/LConn1 -- Ócsa___Zugló_CN_100863542_220000_CN_354667530_220000/LConn1 -- Ócsa___Zugló_CN_100863542_220000_CN_100844170_220000/LConn1
  Detk___Zugló_II__CN_100863542_220000_CN_301002581_220000/LConn2 -- T_100863542__Zugló_alállomás/LConn2 -- Göd___Zugló_CN_100863542_220000_CN_100872886_220000/LConn2 -- Ócsa___Zugló_CN_100863542_220000_CN_354667530_220000/LConn2 -- Ócsa___Zugló_CN_100863542_220000_CN_100844170_220000/LConn2
  Detk___Zugló_II__CN_100863542_220000_CN_301002581_220000/LConn3 -- T_100863542__Zugló_alállomás/LConn3 -- Göd___Zugló_CN_100863542_220000_CN_100872886_220000/LConn3 -- Ócsa___Zugló_CN_100863542_220000_CN_354667530_220000/LConn3 -- Ócsa___Zugló_CN_100863542_220000_CN_100844170_220000/LConn3 -- bus217/LConn1
  T_301002581__/LConn1 -- Detk___Zugló_II__CN_100863542_220000_CN_301002581_220000/RConn1
  T_301002581__/LConn2 -- Detk___Zugló_II__CN_100863542_220000_CN_301002581_220000/RConn2
  Detk___Zugló_II__CN_100863542_220000_CN_301002581_220000/RConn3 -- T_301002581__/LConn3 -- bus218/LConn1
  T_100872886__Göd_alállomás/RConn1 -- Göd___Zugló_CN_100863542_220000_CN_100872886_220000/RConn1
  T_100872886__Göd_alállomás/RConn2 -- Göd___Zugló_CN_100863542_220000_CN_100872886_220000/RConn2
  Göd___Zugló_CN_100863542_220000_CN_100872886_220000/RConn3 -- T_100872886__Göd_alállomás/RConn3 -- bus219/LConn1
  T_354667530__/LConn1 -- Ócsa___Zugló_CN_100863542_220000_CN_354667530_220000/RConn1
  T_354667530__/LConn2 -- Ócsa___Zugló_CN_100863542_220000_CN_354667530_220000/RConn2
  Ócsa___Zugló_CN_100863542_220000_CN_354667530_220000/RConn3 -- T_354667530__/LConn3 -- bus220/LConn1
  Ócsa___Zugló_CN_100863542_220000_CN_100844170_220000/RConn1 -- T_100844170_220000_Ócsai_transzformátor_állomás/LConn1 -- Dunamenti___Ócsa_II__CN_100844170_220000_CN_228355796_120000/RConn1
  Ócsa___Zugló_CN_100863542_220000_CN_100844170_220000/RConn2 -- T_100844170_220000_Ócsai_transzformátor_állomás/LConn2 -- Dunamenti___Ócsa_II__CN_100844170_220000_CN_228355796_120000/RConn2
  Ócsa___Zugló_CN_100863542_220000_CN_100844170_220000/RConn3 -- T_100844170_220000_Ócsai_transzformátor_állomás/LConn3 -- Dunamenti___Ócsa_II__CN_100844170_220000_CN_228355796_120000/RConn3 -- bus221/LConn1
  _CN_100804905_220000_CN_228355796_120000/RConn1 -- T_100804905__Martonvásár_alállomás/RConn1 -- L_100804905/LConn1
  _CN_100804905_220000_CN_228355796_120000/RConn2 -- T_100804905__Martonvásár_alállomás/RConn2 -- L_100804905/LConn2
  _CN_100804905_220000_CN_228355796_120000/RConn3 -- T_100804905__Martonvásár_alállomás/RConn3 -- L_100804905/LConn3 -- bus222/LConn1
  T_104033901_220000;120000;35000;20000;10000_Debrecen_220_120_35_20_10_kV_os_Alállomás/LConn1 -- Sajószöged___Debrecen_CN_104033901_220000_CN_155227474_220000/LConn1
  T_104033901_220000;120000;35000;20000;10000_Debrecen_220_120_35_20_10_kV_os_Alállomás/LConn2 -- Sajószöged___Debrecen_CN_104033901_220000_CN_155227474_220000/LConn2
  Sajószöged___Debrecen_CN_104033901_220000_CN_155227474_220000/LConn3 -- T_104033901_220000;120000;35000;20000;10000_Debrecen_220_120_35_20_10_kV_os_Alállomás/LConn3 -- bus223/LConn1
  Sajószöged___Debrecen_CN_104033901_220000_CN_155227474_220000/RConn1 -- T_155227474__Sajószöged_alállomás/RConn1 -- _CN_155227474_220000_CN_252028146_220000/LConn1
  Sajószöged___Debrecen_CN_104033901_220000_CN_155227474_220000/RConn2 -- T_155227474__Sajószöged_alállomás/RConn2 -- _CN_155227474_220000_CN_252028146_220000/LConn2
  Sajószöged___Debrecen_CN_104033901_220000_CN_155227474_220000/RConn3 -- T_155227474__Sajószöged_alállomás/RConn3 -- _CN_155227474_220000_CN_252028146_220000/LConn3 -- bus224/LConn1
  Sándorfalva___Szeged_CN_111678830_220000_CN_100962927_220000/LConn1 -- T_111678830__Szeged_alállomás/LConn1 -- Szolnok___Szeged_CN_111678830_220000_CN_252028146_220000/LConn1
  Sándorfalva___Szeged_CN_111678830_220000_CN_100962927_220000/LConn2 -- T_111678830__Szeged_alállomás/LConn2 -- Szolnok___Szeged_CN_111678830_220000_CN_252028146_220000/LConn2
  Sándorfalva___Szeged_CN_111678830_220000_CN_100962927_220000/LConn3 -- T_111678830__Szeged_alállomás/LConn3 -- Szolnok___Szeged_CN_111678830_220000_CN_252028146_220000/LConn3 -- bus225/LConn1
  T_100962927__Sándorfalva_alállomás/RConn1 -- Sándorfalva___Szeged_CN_111678830_220000_CN_100962927_220000/RConn1
  T_100962927__Sándorfalva_alállomás/RConn2 -- Sándorfalva___Szeged_CN_111678830_220000_CN_100962927_220000/RConn2
  Sándorfalva___Szeged_CN_111678830_220000_CN_100962927_220000/RConn3 -- T_100962927__Sándorfalva_alállomás/RConn3 -- bus226/LConn1
  Szolnok___Szeged_CN_111678830_220000_CN_252028146_220000/RConn1 -- T_252028146_220000;120000;12000_Szolnok_220_120_20_kV_os_Alállomás/RConn1 -- _CN_155227474_220000_CN_252028146_220000/RConn1
  Szolnok___Szeged_CN_111678830_220000_CN_252028146_220000/RConn2 -- T_252028146_220000;120000;12000_Szolnok_220_120_20_kV_os_Alállomás/RConn2 -- _CN_155227474_220000_CN_252028146_220000/RConn2
  Szolnok___Szeged_CN_111678830_220000_CN_252028146_220000/RConn3 -- T_252028146_220000;120000;12000_Szolnok_220_120_20_kV_os_Alállomás/RConn3 -- _CN_155227474_220000_CN_252028146_220000/RConn3 -- bus227/LConn1
  T_100804921__Dunamenti/LConn1 -- _CN_100804921_220000_CN_228355796_120000/RConn1
  T_100804921__Dunamenti/LConn2 -- _CN_100804921_220000_CN_228355796_120000/RConn2
  _CN_100804921_220000_CN_228355796_120000/RConn3 -- T_100804921__Dunamenti/LConn3 -- bus228/LConn1
  T_195155625__/LConn1 -- Békéscsaba–Nagyvárad_távvezeték_CN_195155625_400000_CN_195168461_400000/LConn1
  T_195155625__/LConn2 -- Békéscsaba–Nagyvárad_távvezeték_CN_195155625_400000_CN_195168461_400000/LConn2
  Békéscsaba–Nagyvárad_távvezeték_CN_195155625_400000_CN_195168461_400000/LConn3 -- T_195155625__/LConn3 -- bus229/LConn1
  Békéscsaba–Nagyvárad_távvezeték_CN_195155625_400000_CN_195168461_400000/RConn1 -- T_195168461__/LConn1 -- Szolnok___Békéscsaba_CN_195168461_400000_CN_252028146_400000/LConn1 -- Sándorfalva___Békéscsaba_CN_195168461_400000_CN_100962927_400000/LConn1
  Békéscsaba–Nagyvárad_távvezeték_CN_195155625_400000_CN_195168461_400000/RConn2 -- T_195168461__/LConn2 -- Szolnok___Békéscsaba_CN_195168461_400000_CN_252028146_400000/LConn2 -- Sándorfalva___Békéscsaba_CN_195168461_400000_CN_100962927_400000/LConn2
  Békéscsaba–Nagyvárad_távvezeték_CN_195155625_400000_CN_195168461_400000/RConn3 -- T_195168461__/LConn3 -- Szolnok___Békéscsaba_CN_195168461_400000_CN_252028146_400000/LConn3 -- Sándorfalva___Békéscsaba_CN_195168461_400000_CN_100962927_400000/LConn3 -- bus230/LConn1
  Győr___Litér_CN_65034002_400000_CN_142106943_400000/LConn1 -- T_65034002_400000;120000_Litér_400_120_kV_alállomás/LConn1 -- Litér–Hévíz_CN_65034002_400000_CN_96705565_400000/LConn1 -- Győr___Litér_CN_65034002_400000_CN_124244078_400000/LConn1 -- _CN_65034002_400000_CN_100788162_400000/LConn1 -- _CN_65034002_400000_CN_113570302_400000/LConn1 -- Litér___Martonvásár_CN_65034002_400000_CN_100804905_400000/LConn1
  Győr___Litér_CN_65034002_400000_CN_142106943_400000/LConn2 -- T_65034002_400000;120000_Litér_400_120_kV_alállomás/LConn2 -- Litér–Hévíz_CN_65034002_400000_CN_96705565_400000/LConn2 -- Győr___Litér_CN_65034002_400000_CN_124244078_400000/LConn2 -- _CN_65034002_400000_CN_100788162_400000/LConn2 -- _CN_65034002_400000_CN_113570302_400000/LConn2 -- Litér___Martonvásár_CN_65034002_400000_CN_100804905_400000/LConn2
  Győr___Litér_CN_65034002_400000_CN_142106943_400000/LConn3 -- T_65034002_400000;120000_Litér_400_120_kV_alállomás/LConn3 -- Litér–Hévíz_CN_65034002_400000_CN_96705565_400000/LConn3 -- bus231/LConn1 -- Győr___Litér_CN_65034002_400000_CN_124244078_400000/LConn3 -- _CN_65034002_400000_CN_100788162_400000/LConn3 -- _CN_65034002_400000_CN_113570302_400000/LConn3 -- Litér___Martonvásár_CN_65034002_400000_CN_100804905_400000/LConn3
  Győr___Litér_CN_65034002_400000_CN_142106943_400000/RConn1 -- T_142106943_400000_Gönyü_400kV_alállomás/LConn1 -- _CN_142106943_400000_CN_350933543_400000/LConn1
  Győr___Litér_CN_65034002_400000_CN_142106943_400000/RConn2 -- T_142106943_400000_Gönyü_400kV_alállomás/LConn2 -- _CN_142106943_400000_CN_350933543_400000/LConn2
  Győr___Litér_CN_65034002_400000_CN_142106943_400000/RConn3 -- T_142106943_400000_Gönyü_400kV_alállomás/LConn3 -- _CN_142106943_400000_CN_350933543_400000/LConn3 -- bus232/LConn1
  Győr___Litér_CN_65034002_400000_CN_124244078_400000/RConn1 -- T_124244078__Győr_Kelet_alállomás/LConn1 -- _CN_124244078_400000_CN_166155511_400000/LConn1
  Győr___Litér_CN_65034002_400000_CN_124244078_400000/RConn2 -- T_124244078__Győr_Kelet_alállomás/LConn2 -- _CN_124244078_400000_CN_166155511_400000/LConn2
  Győr___Litér_CN_65034002_400000_CN_124244078_400000/RConn3 -- T_124244078__Győr_Kelet_alállomás/LConn3 -- _CN_124244078_400000_CN_166155511_400000/LConn3 -- bus233/LConn1
  _CN_65034002_400000_CN_100788162_400000/RConn1 -- T_100788162__Paks_alállomás/LConn1 -- Paks___Sándorfalva_CN_100788162_400000_CN_100962927_400000/LConn1 -- _CN_100788162_400000_CN_110144984_400000/LConn1 -- Paks–Pécs_400_kV_CN_33846555_400000_CN_100788162_400000/LConn1 -- Martonvásár___Paks_400_kV_os_távvezeték_CN_100804905_400000_CN_100788162_400000/LConn1
  _CN_65034002_400000_CN_100788162_400000/RConn2 -- T_100788162__Paks_alállomás/LConn2 -- Paks___Sándorfalva_CN_100788162_400000_CN_100962927_400000/LConn2 -- _CN_100788162_400000_CN_110144984_400000/LConn2 -- Paks–Pécs_400_kV_CN_33846555_400000_CN_100788162_400000/LConn2 -- Martonvásár___Paks_400_kV_os_távvezeték_CN_100804905_400000_CN_100788162_400000/LConn2
  _CN_65034002_400000_CN_100788162_400000/RConn3 -- T_100788162__Paks_alállomás/LConn3 -- Paks___Sándorfalva_CN_100788162_400000_CN_100962927_400000/LConn3 -- _CN_100788162_400000_CN_110144984_400000/LConn3 -- bus234/LConn1 -- Paks–Pécs_400_kV_CN_33846555_400000_CN_100788162_400000/LConn3 -- Martonvásár___Paks_400_kV_os_távvezeték_CN_100804905_400000_CN_100788162_400000/LConn3
  _CN_65034002_400000_CN_113570302_400000/RConn1 -- T_113570302_400000;120000_Toponár_400_120_kV_alállomás/LConn1 -- Hévíz–Toponár_CN_96705565_400000_CN_113570302_400000/LConn1
  _CN_65034002_400000_CN_113570302_400000/RConn2 -- T_113570302_400000;120000_Toponár_400_120_kV_alállomás/LConn2 -- Hévíz–Toponár_CN_96705565_400000_CN_113570302_400000/LConn2
  _CN_65034002_400000_CN_113570302_400000/RConn3 -- T_113570302_400000;120000_Toponár_400_120_kV_alállomás/LConn3 -- Hévíz–Toponár_CN_96705565_400000_CN_113570302_400000/LConn3 -- bus235/LConn1
  Litér___Martonvásár_CN_65034002_400000_CN_100804905_400000/RConn1 -- T_100804905__Martonvásár_alállomás/LConn1 -- _CN_100804905_400000_CN_254847446_400000/LConn1 -- Martonvásár___Paks_400_kV_os_távvezeték_CN_100804905_400000_CN_100788162_400000/RConn1 -- _CN_142109093_400000_CN_100804905_400000/LConn1
  Litér___Martonvásár_CN_65034002_400000_CN_100804905_400000/RConn2 -- T_100804905__Martonvásár_alállomás/LConn2 -- _CN_100804905_400000_CN_254847446_400000/LConn2 -- Martonvásár___Paks_400_kV_os_távvezeték_CN_100804905_400000_CN_100788162_400000/RConn2 -- _CN_142109093_400000_CN_100804905_400000/LConn2
  Litér___Martonvásár_CN_65034002_400000_CN_100804905_400000/RConn3 -- T_100804905__Martonvásár_alállomás/LConn3 -- _CN_100804905_400000_CN_254847446_400000/LConn3 -- Martonvásár___Paks_400_kV_os_távvezeték_CN_100804905_400000_CN_100788162_400000/RConn3 -- bus236/LConn1 -- _CN_142109093_400000_CN_100804905_400000/LConn3
  Litér–Hévíz_CN_65034002_400000_CN_96705565_400000/RConn1 -- T_96705565_400000;120000_Hévíz_400_120_kV_alállomás/LConn1 -- Hévíz–Toponár_CN_96705565_400000_CN_113570302_400000/RConn1 -- Hévíz–Szombathely_CN_96705565_400000_CN_166155511_400000/LConn1
  Litér–Hévíz_CN_65034002_400000_CN_96705565_400000/RConn2 -- T_96705565_400000;120000_Hévíz_400_120_kV_alállomás/LConn2 -- Hévíz–Toponár_CN_96705565_400000_CN_113570302_400000/RConn2 -- Hévíz–Szombathely_CN_96705565_400000_CN_166155511_400000/LConn2
  Litér–Hévíz_CN_65034002_400000_CN_96705565_400000/RConn3 -- T_96705565_400000;120000_Hévíz_400_120_kV_alállomás/LConn3 -- Hévíz–Toponár_CN_96705565_400000_CN_113570302_400000/RConn3 -- Hévíz–Szombathely_CN_96705565_400000_CN_166155511_400000/LConn3 -- bus237/LConn1
  _CN_124244078_400000_CN_166155511_400000/RConn1 -- T_166155511_400000;120000_Szombathely_400_120_kV_alállomás/LConn1 -- Hévíz–Szombathely_CN_96705565_400000_CN_166155511_400000/RConn1
  _CN_124244078_400000_CN_166155511_400000/RConn2 -- T_166155511_400000;120000_Szombathely_400_120_kV_alállomás/LConn2 -- Hévíz–Szombathely_CN_96705565_400000_CN_166155511_400000/RConn2
  _CN_124244078_400000_CN_166155511_400000/RConn3 -- T_166155511_400000;120000_Szombathely_400_120_kV_alállomás/LConn3 -- Hévíz–Szombathely_CN_96705565_400000_CN_166155511_400000/RConn3 -- bus238/LConn1
  T_33846555_400000;120000_Pécs_Kelet_alállomás/LConn1 -- Paks–Pécs_400_kV_CN_33846555_400000_CN_100788162_400000/RConn1
  T_33846555_400000;120000_Pécs_Kelet_alállomás/LConn2 -- Paks–Pécs_400_kV_CN_33846555_400000_CN_100788162_400000/RConn2
  Paks–Pécs_400_kV_CN_33846555_400000_CN_100788162_400000/RConn3 -- T_33846555_400000;120000_Pécs_Kelet_alállomás/LConn3 -- bus239/LConn1
  _CN_142109093_400000_CN_100872886_400000/LConn1 -- T_142109093__Albertirsa_alállomás/LConn1 -- _CN_142109093_400000_CN_100804905_400000/RConn1 -- Szolnok–Albertirsa_CN_142109093_400000_CN_252028146_400000/LConn1
  _CN_142109093_400000_CN_100872886_400000/LConn2 -- T_142109093__Albertirsa_alállomás/LConn2 -- _CN_142109093_400000_CN_100804905_400000/RConn2 -- Szolnok–Albertirsa_CN_142109093_400000_CN_252028146_400000/LConn2
  _CN_142109093_400000_CN_100872886_400000/LConn3 -- T_142109093__Albertirsa_alállomás/LConn3 -- _CN_142109093_400000_CN_100804905_400000/RConn3 -- bus240/LConn1 -- Szolnok–Albertirsa_CN_142109093_400000_CN_252028146_400000/LConn3
  _CN_142109093_400000_CN_100872886_400000/RConn1 -- T_100872886__Göd_alállomás/LConn1 -- Göd___Sajószöged_CN_100872886_400000_CN_155227474_400000/LConn1
  _CN_142109093_400000_CN_100872886_400000/RConn2 -- T_100872886__Göd_alállomás/LConn2 -- Göd___Sajószöged_CN_100872886_400000_CN_155227474_400000/LConn2
  _CN_142109093_400000_CN_100872886_400000/RConn3 -- T_100872886__Göd_alállomás/LConn3 -- Göd___Sajószöged_CN_100872886_400000_CN_155227474_400000/LConn3 -- bus241/LConn1
  Szolnok–Albertirsa_CN_142109093_400000_CN_252028146_400000/RConn1 -- T_252028146_220000;120000;12000_Szolnok_220_120_20_kV_os_Alállomás/LConn1 -- Szolnok___Békéscsaba_CN_195168461_400000_CN_252028146_400000/RConn1
  Szolnok–Albertirsa_CN_142109093_400000_CN_252028146_400000/RConn2 -- T_252028146_220000;120000;12000_Szolnok_220_120_20_kV_os_Alállomás/LConn2 -- Szolnok___Békéscsaba_CN_195168461_400000_CN_252028146_400000/RConn2
  Szolnok–Albertirsa_CN_142109093_400000_CN_252028146_400000/RConn3 -- T_252028146_220000;120000;12000_Szolnok_220_120_20_kV_os_Alállomás/LConn3 -- Szolnok___Békéscsaba_CN_195168461_400000_CN_252028146_400000/RConn3 -- bus242/LConn1
  T_254847446__Bicske_dél_alállomás/LConn1 -- _CN_100804905_400000_CN_254847446_400000/RConn1
  T_254847446__Bicske_dél_alállomás/LConn2 -- _CN_100804905_400000_CN_254847446_400000/RConn2
  _CN_100804905_400000_CN_254847446_400000/RConn3 -- T_254847446__Bicske_dél_alállomás/LConn3 -- bus243/LConn1
  T_167896114__/LConn1 -- _CN_167896114_400000_CN_155803703_400000/LConn1
  T_167896114__/LConn2 -- _CN_167896114_400000_CN_155803703_400000/LConn2
  _CN_167896114_400000_CN_155803703_400000/LConn3 -- T_167896114__/LConn3 -- bus244/LConn1
  _CN_167896114_400000_CN_155803703_400000/RConn1 -- T_155803703__Felsőzsolca_alállomás/LConn1 -- Sajószöged__Felsőzsolca_II__CN_155803703_400000_CN_155227474_400000/LConn1
  _CN_167896114_400000_CN_155803703_400000/RConn2 -- T_155803703__Felsőzsolca_alállomás/LConn2 -- Sajószöged__Felsőzsolca_II__CN_155803703_400000_CN_155227474_400000/LConn2
  _CN_167896114_400000_CN_155803703_400000/RConn3 -- T_155803703__Felsőzsolca_alállomás/LConn3 -- Sajószöged__Felsőzsolca_II__CN_155803703_400000_CN_155227474_400000/LConn3 -- bus245/LConn1
  Göd___Sajószöged_CN_100872886_400000_CN_155227474_400000/RConn1 -- T_155227474__Sajószöged_alállomás/LConn1 -- Sajószöged___Мукачево_(Munkács)_CN_155227474_400000_CN_203815422_400000/LConn1 -- Sajószöged__Felsőzsolca_II__CN_155803703_400000_CN_155227474_400000/RConn1
  Göd___Sajószöged_CN_100872886_400000_CN_155227474_400000/RConn2 -- T_155227474__Sajószöged_alállomás/LConn2 -- Sajószöged___Мукачево_(Munkács)_CN_155227474_400000_CN_203815422_400000/LConn2 -- Sajószöged__Felsőzsolca_II__CN_155803703_400000_CN_155227474_400000/RConn2
  Göd___Sajószöged_CN_100872886_400000_CN_155227474_400000/RConn3 -- T_155227474__Sajószöged_alállomás/LConn3 -- Sajószöged___Мукачево_(Munkács)_CN_155227474_400000_CN_203815422_400000/LConn3 -- bus246/LConn1 -- Sajószöged__Felsőzsolca_II__CN_155803703_400000_CN_155227474_400000/RConn3
  G_350933543_/RConn1 -- _CN_142106943_400000_CN_350933543_400000/RConn1
  G_350933543_/RConn2 -- _CN_142106943_400000_CN_350933543_400000/RConn2
  _CN_142106943_400000_CN_350933543_400000/RConn3 -- G_350933543_/RConn3 -- bus247/LConn1
  Paks___Sándorfalva_CN_100788162_400000_CN_100962927_400000/RConn1 -- T_100962927__Sándorfalva_alállomás/LConn1 -- Sándorfalva___Békéscsaba_CN_195168461_400000_CN_100962927_400000/RConn1 -- Sándorfalva___Arad_CN_101158766_400000_CN_100962927_400000/LConn1 -- Sándorfalva___Subotica_CN_100962927_400000_CN_89109496_400000/LConn1
  Paks___Sándorfalva_CN_100788162_400000_CN_100962927_400000/RConn2 -- T_100962927__Sándorfalva_alállomás/LConn2 -- Sándorfalva___Békéscsaba_CN_195168461_400000_CN_100962927_400000/RConn2 -- Sándorfalva___Arad_CN_101158766_400000_CN_100962927_400000/LConn2 -- Sándorfalva___Subotica_CN_100962927_400000_CN_89109496_400000/LConn2
  Paks___Sándorfalva_CN_100788162_400000_CN_100962927_400000/RConn3 -- T_100962927__Sándorfalva_alállomás/LConn3 -- Sándorfalva___Békéscsaba_CN_195168461_400000_CN_100962927_400000/RConn3 -- Sándorfalva___Arad_CN_101158766_400000_CN_100962927_400000/LConn3 -- Sándorfalva___Subotica_CN_100962927_400000_CN_89109496_400000/LConn3 -- bus248/LConn1
  G_110144984_Paksi_Atomerőmű/RConn1 -- _CN_100788162_400000_CN_110144984_400000/RConn1
  G_110144984_Paksi_Atomerőmű/RConn2 -- _CN_100788162_400000_CN_110144984_400000/RConn2
  _CN_100788162_400000_CN_110144984_400000/RConn3 -- G_110144984_Paksi_Atomerőmű/RConn3 -- bus249/LConn1
  T_203815422_400000;220000;110000;35000_Мукачеве_400/LConn1 -- Sajószöged___Мукачево_(Munkács)_CN_155227474_400000_CN_203815422_400000/RConn1
  T_203815422_400000;220000;110000;35000_Мукачеве_400/LConn2 -- Sajószöged___Мукачево_(Munkács)_CN_155227474_400000_CN_203815422_400000/RConn2
  Sajószöged___Мукачево_(Munkács)_CN_155227474_400000_CN_203815422_400000/RConn3 -- T_203815422_400000;220000;110000;35000_Мукачеве_400/LConn3 -- bus250/LConn1
  T_101158766__/LConn1 -- Sándorfalva___Arad_CN_101158766_400000_CN_100962927_400000/RConn1
  T_101158766__/LConn2 -- Sándorfalva___Arad_CN_101158766_400000_CN_100962927_400000/RConn2
  Sándorfalva___Arad_CN_101158766_400000_CN_100962927_400000/RConn3 -- T_101158766__/LConn3 -- bus251/LConn1
  T_89109496__/LConn1 -- Sándorfalva___Subotica_CN_100962927_400000_CN_89109496_400000/RConn1
  T_89109496__/LConn2 -- Sándorfalva___Subotica_CN_100962927_400000_CN_89109496_400000/RConn2
  Sándorfalva___Subotica_CN_100962927_400000_CN_89109496_400000/RConn3 -- T_89109496__/LConn3 -- bus252/LConn1
  T_38485068__TS_Donji_Miholjac/RConn1 -- L_38485068/LConn1
  T_38485068__TS_Donji_Miholjac/RConn2 -- L_38485068/LConn2
  L_38485068/LConn3 -- T_38485068__TS_Donji_Miholjac/RConn3 -- bus253/LConn1
  T_60222001__Umspannwerk_Frauenkirchen/RConn1 -- L_60222001/LConn1
  T_60222001__Umspannwerk_Frauenkirchen/RConn2 -- L_60222001/LConn2
  L_60222001/LConn3 -- T_60222001__Umspannwerk_Frauenkirchen/RConn3 -- bus254/LConn1
  T_174474431__Umspannwerk_Andau/RConn1 -- L_174474431/LConn1
  T_174474431__Umspannwerk_Andau/RConn2 -- L_174474431/LConn2
  L_174474431/LConn3 -- T_174474431__Umspannwerk_Andau/RConn3 -- bus255/LConn1
  T_144039427__Várpalota_alállomás/RConn1 -- L_144039427/LConn1
  T_144039427__Várpalota_alállomás/RConn2 -- L_144039427/LConn2
  L_144039427/LConn3 -- T_144039427__Várpalota_alállomás/RConn3 -- bus256/LConn1
  T_254910050__Tatabánya_120_kV_alállomás/RConn1 -- L_254910050/LConn1
  T_254910050__Tatabánya_120_kV_alállomás/RConn2 -- L_254910050/LConn2
  L_254910050/LConn3 -- T_254910050__Tatabánya_120_kV_alállomás/RConn3 -- bus257/LConn1
  T_103960070_120000_Angyalföldi/RConn1 -- L_103960070/LConn1
  T_103960070_120000_Angyalföldi/RConn2 -- L_103960070/LConn2
  L_103960070/LConn3 -- T_103960070_120000_Angyalföldi/RConn3 -- bus258/LConn1
  T_103952390_120000_/RConn1 -- L_103952390/LConn1
  T_103952390_120000_/RConn2 -- L_103952390/LConn2
  L_103952390/LConn3 -- T_103952390_120000_/RConn3 -- bus259/LConn1
  T_252610696__/RConn1 -- L_252610696/LConn1
  T_252610696__/RConn2 -- L_252610696/LConn2
  L_252610696/LConn3 -- T_252610696__/RConn3 -- bus260/LConn1
  T_135295847__/RConn1 -- L_135295847/LConn1
  T_135295847__/RConn2 -- L_135295847/LConn2
  L_135295847/LConn3 -- T_135295847__/RConn3 -- bus261/LConn1
  T_104011271__Soroksár_alállomás/RConn1 -- L_104011271/LConn1
  T_104011271__Soroksár_alállomás/RConn2 -- L_104011271/LConn2
  L_104011271/LConn3 -- T_104011271__Soroksár_alállomás/RConn3 -- bus262/LConn1
  T_103965083__Kőbánya_alállomás/RConn1 -- L_103965083/LConn1
  T_103965083__Kőbánya_alállomás/RConn2 -- L_103965083/LConn2
  L_103965083/LConn3 -- T_103965083__Kőbánya_alállomás/RConn3 -- bus263/LConn1
  T_351270546__/RConn1 -- L_351270546/LConn1
  T_351270546__/RConn2 -- L_351270546/LConn2
  L_351270546/LConn3 -- T_351270546__/RConn3 -- bus264/LConn1
  T_103963492_120000_Pestszentlőrinc/RConn1 -- L_103963492/LConn1
  T_103963492_120000_Pestszentlőrinc/RConn2 -- L_103963492/LConn2
  L_103963492/LConn3 -- T_103963492_120000_Pestszentlőrinc/RConn3 -- bus265/LConn1
  T_190281225__Ajka/RConn1 -- L_190281225/LConn1
  T_190281225__Ajka/RConn2 -- L_190281225/LConn2
  L_190281225/LConn3 -- T_190281225__Ajka/RConn3 -- bus266/LConn1
  T_175703168_120000_Sümeg_alállomás/RConn1 -- L_175703168/LConn1
  T_175703168_120000_Sümeg_alállomás/RConn2 -- L_175703168/LConn2
  L_175703168/LConn3 -- T_175703168_120000_Sümeg_alállomás/RConn3 -- bus267/LConn1
  T_107894433__Zalaegerszeg_dél_alállomás/RConn1 -- L_107894433/LConn1
  T_107894433__Zalaegerszeg_dél_alállomás/RConn2 -- L_107894433/LConn2
  L_107894433/LConn3 -- T_107894433__Zalaegerszeg_dél_alállomás/RConn3 -- bus268/LConn1
  T_209328058__Zalaegerszeg_alállomás/RConn1 -- L_209328058/LConn1
  T_209328058__Zalaegerszeg_alállomás/RConn2 -- L_209328058/LConn2
  L_209328058/LConn3 -- T_209328058__Zalaegerszeg_alállomás/RConn3 -- bus269/LConn1
  T_243983151_120000;11000_Keszthely_alállomás/RConn1 -- L_243983151/LConn1
  T_243983151_120000;11000_Keszthely_alállomás/RConn2 -- L_243983151/LConn2
  L_243983151/LConn3 -- T_243983151_120000;11000_Keszthely_alállomás/RConn3 -- bus270/LConn1
  T_167473416__/RConn1 -- L_167473416/LConn1
  T_167473416__/RConn2 -- L_167473416/LConn2
  L_167473416/LConn3 -- T_167473416__/RConn3 -- bus271/LConn1
  T_320532045__Ajka/RConn1 -- L_320532045/LConn1
  T_320532045__Ajka/RConn2 -- L_320532045/LConn2
  L_320532045/LConn3 -- T_320532045__Ajka/RConn3 -- bus272/LConn1
  T_299594250__/RConn1 -- L_299594250/LConn1
  T_299594250__/RConn2 -- L_299594250/LConn2
  L_299594250/LConn3 -- T_299594250__/RConn3 -- bus273/LConn1
  T_299717539__/RConn1 -- L_299717539/LConn1
  T_299717539__/RConn2 -- L_299717539/LConn2
  L_299717539/LConn3 -- T_299717539__/RConn3 -- bus274/LConn1
  T_299717558__Rétság_alállomás/RConn1 -- L_299717558/LConn1
  T_299717558__Rétság_alállomás/RConn2 -- L_299717558/LConn2
  L_299717558/LConn3 -- T_299717558__Rétság_alállomás/RConn3 -- bus275/LConn1
  T_167798796__Nagyatád_alállomás/RConn1 -- L_167798796/LConn1
  T_167798796__Nagyatád_alállomás/RConn2 -- L_167798796/LConn2
  L_167798796/LConn3 -- T_167798796__Nagyatád_alállomás/RConn3 -- bus276/LConn1
  T_31538924__Kaposvár_alállomás/RConn1 -- L_31538924/LConn1
  T_31538924__Kaposvár_alállomás/RConn2 -- L_31538924/LConn2
  L_31538924/LConn3 -- T_31538924__Kaposvár_alállomás/RConn3 -- bus277/LConn1
  T_121241890__Szigetvár_120_kV_alállomás/RConn1 -- L_121241890/LConn1
  T_121241890__Szigetvár_120_kV_alállomás/RConn2 -- L_121241890/LConn2
  L_121241890/LConn3 -- T_121241890__Szigetvár_120_kV_alállomás/RConn3 -- bus278/LConn1
  T_244495956__Csurgó_alállomás/RConn1 -- L_244495956/LConn1
  T_244495956__Csurgó_alállomás/RConn2 -- L_244495956/LConn2
  L_244495956/LConn3 -- T_244495956__Csurgó_alállomás/RConn3 -- bus279/LConn1
  T_203404634_120000;20000;10000_Nagykanizsa_alállomás/RConn1 -- L_203404634/LConn1
  T_203404634_120000;20000;10000_Nagykanizsa_alállomás/RConn2 -- L_203404634/LConn2
  L_203404634/LConn3 -- T_203404634_120000;20000;10000_Nagykanizsa_alállomás/RConn3 -- bus280/LConn1
  T_254851597__Bicske_alállomás/RConn1 -- L_254851597/LConn1
  T_254851597__Bicske_alállomás/RConn2 -- L_254851597/LConn2
  L_254851597/LConn3 -- T_254851597__Bicske_alállomás/RConn3 -- bus281/LConn1
  T_350686736__Győr_Dunapart_alállomás/RConn1 -- L_350686736/LConn1
  T_350686736__Győr_Dunapart_alállomás/RConn2 -- L_350686736/LConn2
  L_350686736/LConn3 -- T_350686736__Győr_Dunapart_alállomás/RConn3 -- bus282/LConn1
  T_350230665__Győr_ÉDÁSZ_alállomás/RConn1 -- L_350230665/LConn1
  T_350230665__Győr_ÉDÁSZ_alállomás/RConn2 -- L_350230665/LConn2
  L_350230665/LConn3 -- T_350230665__Győr_ÉDÁSZ_alállomás/RConn3 -- bus283/LConn1
  T_288399377__Szeged_Cserepes_sori_alállomás/RConn1 -- L_288399377/LConn1
  T_288399377__Szeged_Cserepes_sori_alállomás/RConn2 -- L_288399377/LConn2
  L_288399377/LConn3 -- T_288399377__Szeged_Cserepes_sori_alállomás/RConn3 -- bus284/LConn1
  T_296680978__/RConn1 -- L_296680978/LConn1
  T_296680978__/RConn2 -- L_296680978/LConn2
  L_296680978/LConn3 -- T_296680978__/RConn3 -- bus285/LConn1
  T_119367515__/RConn1 -- L_119367515/LConn1
  T_119367515__/RConn2 -- L_119367515/LConn2
  L_119367515/LConn3 -- T_119367515__/RConn3 -- bus286/LConn1
  T_251991299_220000;120000_Detk_220_120_kV_os_alállomás/RConn1 -- L_251991299/LConn1
  T_251991299_220000;120000_Detk_220_120_kV_os_alállomás/RConn2 -- L_251991299/LConn2
  L_251991299/LConn3 -- T_251991299_220000;120000_Detk_220_120_kV_os_alállomás/RConn3 -- bus287/LConn1
  T_173757619__Nagybátony_alállomás/RConn1 -- L_173757619/LConn1
  T_173757619__Nagybátony_alállomás/RConn2 -- L_173757619/LConn2
  L_173757619/LConn3 -- T_173757619__Nagybátony_alállomás/RConn3 -- bus288/LConn1
  T_299574805__/RConn1 -- L_299574805/LConn1
  T_299574805__/RConn2 -- L_299574805/LConn2
  L_299574805/LConn3 -- T_299574805__/RConn3 -- bus289/LConn1
  T_351673886__/RConn1 -- L_351673886/LConn1
  T_351673886__/RConn2 -- L_351673886/LConn2
  L_351673886/LConn3 -- T_351673886__/RConn3 -- bus290/LConn1
  T_313889220__Kővágószőlős_alállomás/RConn1 -- L_313889220/LConn1
  T_313889220__Kővágószőlős_alállomás/RConn2 -- L_313889220/LConn2
  L_313889220/LConn3 -- T_313889220__Kővágószőlős_alállomás/RConn3 -- bus291/LConn1
  T_285317363__/RConn1 -- L_285317363/LConn1
  T_285317363__/RConn2 -- L_285317363/LConn2
  L_285317363/LConn3 -- T_285317363__/RConn3 -- bus292/LConn1
  T_281553159__Tiszakécske/RConn1 -- L_281553159/LConn1
  T_281553159__Tiszakécske/RConn2 -- L_281553159/LConn2
  L_281553159/LConn3 -- T_281553159__Tiszakécske/RConn3 -- bus293/LConn1
  T_153827138__Városföld_alállomás/RConn1 -- L_153827138/LConn1
  T_153827138__Városföld_alállomás/RConn2 -- L_153827138/LConn2
  L_153827138/LConn3 -- T_153827138__Városföld_alállomás/RConn3 -- bus294/LConn1
  T_289183579__/RConn1 -- L_289183579/LConn1
  T_289183579__/RConn2 -- L_289183579/LConn2
  L_289183579/LConn3 -- T_289183579__/RConn3 -- bus295/LConn1
  T_289183615__/RConn1 -- L_289183615/LConn1
  T_289183615__/RConn2 -- L_289183615/LConn2
  L_289183615/LConn3 -- T_289183615__/RConn3 -- bus296/LConn1
  T_288863087__Mezőtúr_120_kV_alállomás/RConn1 -- L_288863087/LConn1
  T_288863087__Mezőtúr_120_kV_alállomás/RConn2 -- L_288863087/LConn2
  L_288863087/LConn3 -- T_288863087__Mezőtúr_120_kV_alállomás/RConn3 -- bus297/LConn1
  T_121661769_120000_/RConn1 -- L_121661769/LConn1
  T_121661769_120000_/RConn2 -- L_121661769/LConn2
  L_121661769/LConn3 -- T_121661769_120000_/RConn3 -- bus298/LConn1
  T_136396751__Hüvösvölgy_alállomás/RConn1 -- L_136396751/LConn1
  T_136396751__Hüvösvölgy_alállomás/RConn2 -- L_136396751/LConn2
  L_136396751/LConn3 -- T_136396751__Hüvösvölgy_alállomás/RConn3 -- bus299/LConn1
  T_252727452_120000_Pomáz/RConn1 -- L_252727452/LConn1
  T_252727452_120000_Pomáz/RConn2 -- L_252727452/LConn2
  L_252727452/LConn3 -- T_252727452_120000_Pomáz/RConn3 -- bus300/LConn1
  T_116801424_120000_Békásmegyer/RConn1 -- L_116801424/LConn1
  T_116801424_120000_Békásmegyer/RConn2 -- L_116801424/LConn2
  L_116801424/LConn3 -- T_116801424_120000_Békásmegyer/RConn3 -- bus301/LConn1
  T_180089895__Celldömölk/RConn1 -- L_180089895/LConn1
  T_180089895__Celldömölk/RConn2 -- L_180089895/LConn2
  L_180089895/LConn3 -- T_180089895__Celldömölk/RConn3 -- bus302/LConn1
  T_302056631__Ikervár_alállomás/RConn1 -- L_302056631/LConn1
  T_302056631__Ikervár_alállomás/RConn2 -- L_302056631/LConn2
  L_302056631/LConn3 -- T_302056631__Ikervár_alállomás/RConn3 -- bus303/LConn1
  T_245836377_120000_Szombathely_120_kV_alállomás/RConn1 -- L_245836377/LConn1
  T_245836377_120000_Szombathely_120_kV_alállomás/RConn2 -- L_245836377/LConn2
  L_245836377/LConn3 -- T_245836377_120000_Szombathely_120_kV_alállomás/RConn3 -- bus304/LConn1
  T_292353065__MÁV_120_25kV/RConn1 -- L_292353065/LConn1
  T_292353065__MÁV_120_25kV/RConn2 -- L_292353065/LConn2
  L_292353065/LConn3 -- T_292353065__MÁV_120_25kV/RConn3 -- bus305/LConn1
  T_292353077__Simai_úti_120_20kV/RConn1 -- L_292353077/LConn1
  T_292353077__Simai_úti_120_20kV/RConn2 -- L_292353077/LConn2
  L_292353077/LConn3 -- T_292353077__Simai_úti_120_20kV/RConn3 -- bus306/LConn1
  T_229990586_120000;10000_Nyíregyháza_Dél/RConn1 -- L_229990586/LConn1
  T_229990586_120000;10000_Nyíregyháza_Dél/RConn2 -- L_229990586/LConn2
  L_229990586/LConn3 -- T_229990586_120000;10000_Nyíregyháza_Dél/RConn3 -- bus307/LConn1
  T_250030343__Ibrány/RConn1 -- L_250030343/LConn1
  T_250030343__Ibrány/RConn2 -- L_250030343/LConn2
  L_250030343/LConn3 -- T_250030343__Ibrány/RConn3 -- bus308/LConn1
  T_302192173__/RConn1 -- L_302192173/LConn1
  T_302192173__/RConn2 -- L_302192173/LConn2
  L_302192173/LConn3 -- T_302192173__/RConn3 -- bus309/LConn1
  T_293373698__Pécs_Újmecsekalja_alállomás/RConn1 -- L_293373698/LConn1
  T_293373698__Pécs_Újmecsekalja_alállomás/RConn2 -- L_293373698/LConn2
  L_293373698/LConn3 -- T_293373698__Pécs_Újmecsekalja_alállomás/RConn3 -- bus310/LConn1
  T_254787562__Pécs_Kertváros_alállomás/RConn1 -- L_254787562/LConn1
  T_254787562__Pécs_Kertváros_alállomás/RConn2 -- L_254787562/LConn2
  L_254787562/LConn3 -- T_254787562__Pécs_Kertváros_alállomás/RConn3 -- bus311/LConn1
  T_315953570__/RConn1 -- L_315953570/LConn1
  T_315953570__/RConn2 -- L_315953570/LConn2
  L_315953570/LConn3 -- T_315953570__/RConn3 -- bus312/LConn1
  T_121501391__Komló_alállomás/RConn1 -- L_121501391/LConn1
  T_121501391__Komló_alállomás/RConn2 -- L_121501391/LConn2
  L_121501391/LConn3 -- T_121501391__Komló_alállomás/RConn3 -- bus313/LConn1
  T_336632820__Szekszárd_alállomás/RConn1 -- L_336632820/LConn1
  T_336632820__Szekszárd_alállomás/RConn2 -- L_336632820/LConn2
  L_336632820/LConn3 -- T_336632820__Szekszárd_alállomás/RConn3 -- bus314/LConn1
  T_331140850__Pécs_Kelet_alállomás/RConn1 -- L_331140850/LConn1
  T_331140850__Pécs_Kelet_alállomás/RConn2 -- L_331140850/LConn2
  L_331140850/LConn3 -- T_331140850__Pécs_Kelet_alállomás/RConn3 -- bus315/LConn1
  T_156193065__Mohács_120_kV_alállomás/RConn1 -- L_156193065/LConn1
  T_156193065__Mohács_120_kV_alállomás/RConn2 -- L_156193065/LConn2
  L_156193065/LConn3 -- T_156193065__Mohács_120_kV_alállomás/RConn3 -- bus316/LConn1
  T_302192175__Győr_Dél_alállomás/RConn1 -- L_302192175/LConn1
  T_302192175__Győr_Dél_alállomás/RConn2 -- L_302192175/LConn2
  L_302192175/LConn3 -- T_302192175__Győr_Dél_alállomás/RConn3 -- bus317/LConn1
  T_206353058__Károlyháza_alállomás/RConn1 -- L_206353058/LConn1
  T_206353058__Károlyháza_alállomás/RConn2 -- L_206353058/LConn2
  L_206353058/LConn3 -- T_206353058__Károlyháza_alállomás/RConn3 -- bus318/LConn1
  T_302192176__Mosonmagyaróvár_alállomás/RConn1 -- L_302192176/LConn1
  T_302192176__Mosonmagyaróvár_alállomás/RConn2 -- L_302192176/LConn2
  L_302192176/LConn3 -- T_302192176__Mosonmagyaróvár_alállomás/RConn3 -- bus319/LConn1
  T_155021873__Kiskundorozsma_alállomás/RConn1 -- L_155021873/LConn1
  T_155021873__Kiskundorozsma_alállomás/RConn2 -- L_155021873/LConn2
  L_155021873/LConn3 -- T_155021873__Kiskundorozsma_alállomás/RConn3 -- bus320/LConn1
  T_284549184__Kiskunhalas/RConn1 -- L_284549184/LConn1
  T_284549184__Kiskunhalas/RConn2 -- L_284549184/LConn2
  L_284549184/LConn3 -- T_284549184__Kiskunhalas/RConn3 -- bus321/LConn1
  T_296112525__/RConn1 -- L_296112525/LConn1
  T_296112525__/RConn2 -- L_296112525/LConn2
  L_296112525/LConn3 -- T_296112525__/RConn3 -- bus322/LConn1
  T_296944282__/RConn1 -- L_296944282/LConn1
  T_296944282__/RConn2 -- L_296944282/LConn2
  L_296944282/LConn3 -- T_296944282__/RConn3 -- bus323/LConn1
  T_354875849__/RConn1 -- L_354875849/LConn1
  T_354875849__/RConn2 -- L_354875849/LConn2
  L_354875849/LConn3 -- T_354875849__/RConn3 -- bus324/LConn1
  T_304275625__/RConn1 -- L_304275625/LConn1
  T_304275625__/RConn2 -- L_304275625/LConn2
  L_304275625/LConn3 -- T_304275625__/RConn3 -- bus325/LConn1
  T_285825715_120000;20000_Nádudvar_120_20_kV_alállomás/RConn1 -- L_285825715/LConn1
  T_285825715_120000;20000_Nádudvar_120_20_kV_alállomás/RConn2 -- L_285825715/LConn2
  L_285825715/LConn3 -- T_285825715_120000;20000_Nádudvar_120_20_kV_alállomás/RConn3 -- bus326/LConn1
  T_256857667__Püspökladány_120_kV_alállomás/RConn1 -- L_256857667/LConn1
  T_256857667__Püspökladány_120_kV_alállomás/RConn2 -- L_256857667/LConn2
  L_256857667/LConn3 -- T_256857667__Püspökladány_120_kV_alállomás/RConn3 -- bus327/LConn1
  T_204662161_120000;20000_Berettyóújfalu_120_20_kV_alállomás/RConn1 -- L_204662161/LConn1
  T_204662161_120000;20000_Berettyóújfalu_120_20_kV_alállomás/RConn2 -- L_204662161/LConn2
  L_204662161/LConn3 -- T_204662161_120000;20000_Berettyóújfalu_120_20_kV_alállomás/RConn3 -- bus328/LConn1
  T_251018027_220000;120000_Tiszalök_220_120_kV_alállomás/RConn1 -- L_251018027/LConn1
  T_251018027_220000;120000_Tiszalök_220_120_kV_alállomás/RConn2 -- L_251018027/LConn2
  L_251018027/LConn3 -- T_251018027_220000;120000_Tiszalök_220_120_kV_alállomás/RConn3 -- bus329/LConn1
  T_103977434__/RConn1 -- L_103977434/LConn1
  T_103977434__/RConn2 -- L_103977434/LConn2
  L_103977434/LConn3 -- T_103977434__/RConn3 -- bus330/LConn1
  T_297281902__/RConn1 -- L_297281902/LConn1
  T_297281902__/RConn2 -- L_297281902/LConn2
  L_297281902/LConn3 -- T_297281902__/RConn3 -- bus331/LConn1
  T_284478605__/RConn1 -- L_284478605/LConn1
  T_284478605__/RConn2 -- L_284478605/LConn2
  L_284478605/LConn3 -- T_284478605__/RConn3 -- bus332/LConn1
  T_288864314__/RConn1 -- L_288864314/LConn1
  T_288864314__/RConn2 -- L_288864314/LConn2
  L_288864314/LConn3 -- T_288864314__/RConn3 -- bus333/LConn1
  T_289011848__/RConn1 -- L_289011848/LConn1
  T_289011848__/RConn2 -- L_289011848/LConn2
  L_289011848/LConn3 -- T_289011848__/RConn3 -- bus334/LConn1
  T_104027708__Gödöllő_alállomás/RConn1 -- L_104027708/LConn1
  T_104027708__Gödöllő_alállomás/RConn2 -- L_104027708/LConn2
  L_104027708/LConn3 -- T_104027708__Gödöllő_alállomás/RConn3 -- bus335/LConn1
  T_311788819__Siófok_alállomás/RConn1 -- L_311788819/LConn1
  T_311788819__Siófok_alállomás/RConn2 -- L_311788819/LConn2
  L_311788819/LConn3 -- T_311788819__Siófok_alállomás/RConn3 -- bus336/LConn1
  T_311788820__Szőlőskislak_alállomás/RConn1 -- L_311788820/LConn1
  T_311788820__Szőlőskislak_alállomás/RConn2 -- L_311788820/LConn2
  L_311788820/LConn3 -- T_311788820__Szőlőskislak_alállomás/RConn3 -- bus337/LConn1
  T_272940764__/RConn1 -- L_272940764/LConn1
  T_272940764__/RConn2 -- L_272940764/LConn2
  L_272940764/LConn3 -- T_272940764__/RConn3 -- bus338/LConn1
  T_239120448__Lenti_alállomás/RConn1 -- L_239120448/LConn1
  T_239120448__Lenti_alállomás/RConn2 -- L_239120448/LConn2
  L_239120448/LConn3 -- T_239120448__Lenti_alállomás/RConn3 -- bus339/LConn1
  T_243816689__Söjtör_alállomás/RConn1 -- L_243816689/LConn1
  T_243816689__Söjtör_alállomás/RConn2 -- L_243816689/LConn2
  L_243816689/LConn3 -- T_243816689__Söjtör_alállomás/RConn3 -- bus340/LConn1
  T_303049651__Szentgotthárd_alállomás/RConn1 -- L_303049651/LConn1
  T_303049651__Szentgotthárd_alállomás/RConn2 -- L_303049651/LConn2
  L_303049651/LConn3 -- T_303049651__Szentgotthárd_alállomás/RConn3 -- bus341/LConn1
  T_244527955__Pankasz_alállomás/RConn1 -- L_244527955/LConn1
  T_244527955__Pankasz_alállomás/RConn2 -- L_244527955/LConn2
  L_244527955/LConn3 -- T_244527955__Pankasz_alállomás/RConn3 -- bus342/LConn1
  T_156269125__/RConn1 -- L_156269125/LConn1
  T_156269125__/RConn2 -- L_156269125/LConn2
  L_156269125/LConn3 -- T_156269125__/RConn3 -- bus343/LConn1
  T_267155016__Győr_Nádorváros_alállomás/RConn1 -- L_267155016/LConn1
  T_267155016__Győr_Nádorváros_alállomás/RConn2 -- L_267155016/LConn2
  L_267155016/LConn3 -- T_267155016__Győr_Nádorváros_alállomás/RConn3 -- bus344/LConn1
  T_290158092__/RConn1 -- L_290158092/LConn1
  T_290158092__/RConn2 -- L_290158092/LConn2
  L_290158092/LConn3 -- T_290158092__/RConn3 -- bus345/LConn1
  T_311977547__/RConn1 -- L_311977547/LConn1
  T_311977547__/RConn2 -- L_311977547/LConn2
  L_311977547/LConn3 -- T_311977547__/RConn3 -- bus346/LConn1
  T_311977556__/RConn1 -- L_311977556/LConn1
  T_311977556__/RConn2 -- L_311977556/LConn2
  L_311977556/LConn3 -- T_311977556__/RConn3 -- bus347/LConn1
  T_301495268__Kisigmánd_szélerőmű_alállomás/RConn1 -- L_301495268/LConn1
  T_301495268__Kisigmánd_szélerőmű_alállomás/RConn2 -- L_301495268/LConn2
  L_301495268/LConn3 -- T_301495268__Kisigmánd_szélerőmű_alállomás/RConn3 -- bus348/LConn1
  T_248973389__/RConn1 -- L_248973389/LConn1
  T_248973389__/RConn2 -- L_248973389/LConn2
  L_248973389/LConn3 -- T_248973389__/RConn3 -- bus349/LConn1
  T_203076074__Felsőbabád_alállomás/RConn1 -- L_203076074/LConn1
  T_203076074__Felsőbabád_alállomás/RConn2 -- L_203076074/LConn2
  L_203076074/LConn3 -- T_203076074__Felsőbabád_alállomás/RConn3 -- bus350/LConn1
  T_398994184__/RConn1 -- L_398994184/LConn1
  T_398994184__/RConn2 -- L_398994184/LConn2
  L_398994184/LConn3 -- T_398994184__/RConn3 -- bus351/LConn1
  T_315669517__MÁV_Kaposfüred_alállomás/RConn1 -- L_315669517/LConn1
  T_315669517__MÁV_Kaposfüred_alállomás/RConn2 -- L_315669517/LConn2
  L_315669517/LConn3 -- T_315669517__MÁV_Kaposfüred_alállomás/RConn3 -- bus352/LConn1
  T_253313106_120000_/RConn1 -- L_253313106/LConn1
  T_253313106_120000_/RConn2 -- L_253313106/LConn2
  L_253313106/LConn3 -- T_253313106_120000_/RConn3 -- bus353/LConn1
  T_253313109_120000_/RConn1 -- L_253313109/LConn1
  T_253313109_120000_/RConn2 -- L_253313109/LConn2
  L_253313109/LConn3 -- T_253313109_120000_/RConn3 -- bus354/LConn1
  T_253272731_120000_/RConn1 -- L_253272731/LConn1
  T_253272731_120000_/RConn2 -- L_253272731/LConn2
  L_253272731/LConn3 -- T_253272731_120000_/RConn3 -- bus355/LConn1
  T_281841238__Lábatlan_alállomás/RConn1 -- L_281841238/LConn1
  T_281841238__Lábatlan_alállomás/RConn2 -- L_281841238/LConn2
  L_281841238/LConn3 -- T_281841238__Lábatlan_alállomás/RConn3 -- bus356/LConn1
  T_254916093__Tata_alállomás/RConn1 -- L_254916093/LConn1
  T_254916093__Tata_alállomás/RConn2 -- L_254916093/LConn2
  L_254916093/LConn3 -- T_254916093__Tata_alállomás/RConn3 -- bus357/LConn1
  T_209157413_120000_Dorog_alállomás/RConn1 -- L_209157413/LConn1
  T_209157413_120000_Dorog_alállomás/RConn2 -- L_209157413/LConn2
  L_209157413/LConn3 -- T_209157413_120000_Dorog_alállomás/RConn3 -- bus358/LConn1
  T_204596172_120000_Szombathely_Szőlős_alállomás/RConn1 -- L_204596172/LConn1
  T_204596172_120000_Szombathely_Szőlős_alállomás/RConn2 -- L_204596172/LConn2
  L_204596172/LConn3 -- T_204596172_120000_Szombathely_Szőlős_alállomás/RConn3 -- bus359/LConn1
  T_178641777_120000;35000;20000_Sopronkövesd_E_ON_ÉDÁSZ_120_35_20_kV_alállomás/RConn1 -- L_178641777/LConn1
  T_178641777_120000;35000;20000_Sopronkövesd_E_ON_ÉDÁSZ_120_35_20_kV_alállomás/RConn2 -- L_178641777/LConn2
  L_178641777/LConn3 -- T_178641777_120000;35000;20000_Sopronkövesd_E_ON_ÉDÁSZ_120_35_20_kV_alállomás/RConn3 -- bus360/LConn1
  T_312831631__Körmend_alállomás/RConn1 -- L_312831631/LConn1
  T_312831631__Körmend_alállomás/RConn2 -- L_312831631/LConn2
  L_312831631/LConn3 -- T_312831631__Körmend_alállomás/RConn3 -- bus361/LConn1
  T_287791196__/RConn1 -- L_287791196/LConn1
  T_287791196__/RConn2 -- L_287791196/LConn2
  L_287791196/LConn3 -- T_287791196__/RConn3 -- bus362/LConn1
  T_113717515__Békéscsaba_120_kV_alállomás/RConn1 -- L_113717515/LConn1
  T_113717515__Békéscsaba_120_kV_alállomás/RConn2 -- L_113717515/LConn2
  L_113717515/LConn3 -- T_113717515__Békéscsaba_120_kV_alállomás/RConn3 -- bus363/LConn1
  T_287647848__/RConn1 -- L_287647848/LConn1
  T_287647848__/RConn2 -- L_287647848/LConn2
  L_287647848/LConn3 -- T_287647848__/RConn3 -- bus364/LConn1
  T_321513575__Ipari_Park_alállomás/RConn1 -- L_321513575/LConn1
  T_321513575__Ipari_Park_alállomás/RConn2 -- L_321513575/LConn2
  L_321513575/LConn3 -- T_321513575__Ipari_Park_alállomás/RConn3 -- bus365/LConn1
  T_282182285__/RConn1 -- L_282182285/LConn1
  T_282182285__/RConn2 -- L_282182285/LConn2
  L_282182285/LConn3 -- T_282182285__/RConn3 -- bus366/LConn1
  T_234435878__Aszófő_alállomás/RConn1 -- L_234435878/LConn1
  T_234435878__Aszófő_alállomás/RConn2 -- L_234435878/LConn2
  L_234435878/LConn3 -- T_234435878__Aszófő_alállomás/RConn3 -- bus367/LConn1
  T_170160989__Tapolca_alállomás/RConn1 -- L_170160989/LConn1
  T_170160989__Tapolca_alállomás/RConn2 -- L_170160989/LConn2
  L_170160989/LConn3 -- T_170160989__Tapolca_alállomás/RConn3 -- bus368/LConn1
  T_117853438__/RConn1 -- L_117853438/LConn1
  T_117853438__/RConn2 -- L_117853438/LConn2
